simulink model "SimulinkFullblock"  (R2019b)
settings: Solver=VariableStepAuto  StartTime=0.0  StopTime=10  RelTol=1e-3
(part 2 of 5)

== matlab function SimulinkFullblock/Forward Acceleration  ==
  data: q input; pdd output; qd input; qdd input
function pdd    = fcn(q,qd,qdd)
q1= q(1);
q2= q(2);
q3= q(3);
q4= q(4);
q5= q(5);
q6= q(6);
q1d=qd(1);
q2d=qd(2);
q3d=qd(3);
q4d=qd(4);
q5d=qd(5);
q6d=qd(6);
q1dd= qdd(1);
q2dd= qdd(2);
q3dd= qdd(3);
q4dd= qdd(4);
q5dd= qdd(5);
q6dd= qdd(6);
L1=10;
L2=10;
L3=10;
L4=10;

Jdev= [ conj(L4)*(sin(0.0175*conj(q5) + 1.5708)*(0.0175*conj(q1d)*sin(0.0175*conj(q1) - 1.5708)*sin(0.0175*conj(q4) + 1.5708) - 0.0175*cos(0.0175*conj(q1) - 1.5708)*cos(0.0175*conj(q4) + 1.5708)*conj(q4d) - 0.0175*cos(0.0175*conj(q1) - 1.5708)*cos(0.0175*conj(q2) - 1.5708)*cos(0.0175*conj(q4) + 1.5708)*conj(q1d) + 0.0175*cos(0.0175*conj(q4) + 1.5708)*conj(q2d)*sin(0.0175*conj(q1) - 1.5708)*sin(0.0175*conj(q2) - 1.5708) + 0.0175*cos(0.0175*conj(q2) - 1.5708)*conj(q4d)*sin(0.0175*conj(q1) - 1.5708)*sin(0.0175*conj(q4) + 1.5708)) - 0.0175*cos(0.0175*conj(q5) + 1.5708)*conj(q5d)*(cos(0.0175*conj(q1) - 1.5708)*sin(0.0175*conj(q4) + 1.5708) + cos(0.0175*conj(q2) - 1.5708)*cos(0.0175*conj(q4) + 1.5708)*sin(0.0175*conj(q1) - 1.5708)) + 0.0175*cos(0.0175*conj(q1) - 1.5708)*cos(0.0175*conj(q5) + 1.5708)*conj(q1d)*sin(0.0175*conj(q2) - 1.5708) + 0.0175*cos(0.0175*conj(q2) - 1.5708)*cos(0.0175*conj(q5) + 1.5708)*conj(q2d)*sin(0.0175*conj(q1) - 1.5708) - 0.0175*conj(q5d)*sin(0.0175*conj(q1) - 1.5708)*sin(0.0175*conj(q2) - 1.5708)*sin(0.0175*conj(q5) + 1.5708)) - conj(q3d)*sin(0.0175*conj(q1) - 1.5708)*sin(0.0175*conj(q2) - 1.5708) - 0.0175*cos(0.0175*conj(q1) - 1.5708)*conj(q1d)*sin(0.0175*conj(q2) - 1.5708)*(conj(q3) + conj(L2)) - 0.0175*cos(0.0175*conj(q2) - 1.5708)*conj(q2d)*sin(0.0175*conj(q1) - 1.5708)*(conj(q3) + conj(L2)) - 0.0175*cos(0.0175*conj(q1) - 1.5708)*conj(q1d)*sin(0.0175*conj(q2) - 1.5708)*conj(L3) - 0.0175*cos(0.0175*conj(q2) - 1.5708)*conj(q2d)*sin(0.0175*conj(q1) - 1.5708)*conj(L3),                                                                                                                                                                                                                                                                                                                                                                                                                                                                                                                                                                                                                                                                                                                                                                                                                                                                                                                                                                                                                                                                                                                                                                                                                                                                                                                                                                                                                                                                                                                                                                                                                                                                                                                                                                                                                                                                                                                                                                                                                                                                                                                                                                                                                                                                                                                                                                                                                                                                                                                                                                                                                                                                                                                                                                                                                                                                                                                                                                                                                                                                                                                                                                                                                                                                                                                                                                                                                                                                                                                                                                                                                                                                                               cos(0.0175*conj(q1) - 1.5708)*(cos(0.0175*conj(q2) - 1.5708)*conj(q3d) + conj(L4)*(0.0175*cos(0.0175*conj(q5) + 1.5708)*conj(q2d)*sin(0.0175*conj(q2) - 1.5708) + 0.0175*cos(0.0175*conj(q2) - 1.5708)*conj(q5d)*sin(0.0175*conj(q5) + 1.5708) - 0.0175*cos(0.0175*conj(q2) - 1.5708)*cos(0.0175*conj(q4) + 1.5708)*conj(q2d)*sin(0.0175*conj(q5) + 1.5708) - 0.0175*cos(0.0175*conj(q4) + 1.5708)*cos(0.0175*conj(q5) + 1.5708)*conj(q5d)*sin(0.0175*conj(q2) - 1.5708) + 0.0175*conj(q4d)*sin(0.0175*conj(q2) - 1.5708)*sin(0.0175*conj(q4) + 1.5708)*sin(0.0175*conj(q5) + 1.5708)) - 0.0175*conj(q2d)*sin(0.0175*conj(q2) - 1.5708)*conj(L3) - 0.0175*conj(q2d)*sin(0.0175*conj(q2) - 1.5708)*(conj(q3) + conj(L2))) - 0.0175*conj(q1d)*sin(0.0175*conj(q1) - 1.5708)*(cos(0.0175*conj(q2) - 1.5708)*conj(L3) - conj(L4)*(cos(0.0175*conj(q2) - 1.5708)*cos(0.0175*conj(q5) + 1.5708) + cos(0.0175*conj(q4) + 1.5708)*sin(0.0175*conj(q2) - 1.5708)*sin(0.0175*conj(q5) + 1.5708)) + cos(0.0175*conj(q2) - 1.5708)*(conj(q3) + conj(L2))), 0.0175*cos(0.0175*q1 - 1.5708)*cos(0.0175*q2 - 1.5708)*q2d - 0.0175*sin(0.0175*q1 - 1.5708)*sin(0.0175*q2 - 1.5708)*q1d,                                                                                                                                                                                                                                                                                                                                                                                                                                                                                                                                                                                                                                                                                                                                                                                                                                                                                                                                                                                                                                                                                                                                                                                                                                                                                                                                                                                                                                                                                                                                                                                                                                                                                                                                                                                                                                                                                                                                                                                                                                                                                                                                                                                                                                                                                                                                                                                                                                                                          sin(0.0175*conj(q1) - 1.5708)*sin(0.0175*conj(q2) - 1.5708)*(cos(0.0175*conj(q2) - 1.5708)*conj(q3d) - cos(0.0175*conj(q2) - 1.5708)*conj(q3d) + conj(L4)*(0.0175*cos(0.0175*conj(q5) + 1.5708)*conj(q2d)*sin(0.0175*conj(q2) - 1.5708) + 0.0175*cos(0.0175*conj(q2) - 1.5708)*conj(q5d)*sin(0.0175*conj(q5) + 1.5708) - 0.0175*cos(0.0175*conj(q2) - 1.5708)*cos(0.0175*conj(q4) + 1.5708)*conj(q2d)*sin(0.0175*conj(q5) + 1.5708) - 0.0175*cos(0.0175*conj(q4) + 1.5708)*cos(0.0175*conj(q5) + 1.5708)*conj(q5d)*sin(0.0175*conj(q2) - 1.5708) + 0.0175*conj(q4d)*sin(0.0175*conj(q2) - 1.5708)*sin(0.0175*conj(q4) + 1.5708)*sin(0.0175*conj(q5) + 1.5708)) - 0.0175*conj(q2d)*sin(0.0175*conj(q2) - 1.5708)*conj(L3) - 0.0175*conj(q2d)*sin(0.0175*conj(q2) - 1.5708)*(conj(q3) + conj(L2)) + 0.0175*conj(q2d)*sin(0.0175*conj(q2) - 1.5708)*(conj(q3) + conj(L2))) - cos(0.0175*conj(q2) - 1.5708)*(conj(q3d)*sin(0.0175*conj(q1) - 1.5708)*sin(0.0175*conj(q2) - 1.5708) - conj(L4)*(sin(0.0175*conj(q5) + 1.5708)*(0.0175*conj(q1d)*sin(0.0175*conj(q1) - 1.5708)*sin(0.0175*conj(q4) + 1.5708) - 0.0175*cos(0.0175*conj(q1) - 1.5708)*cos(0.0175*conj(q4) + 1.5708)*conj(q4d) - 0.0175*cos(0.0175*conj(q1) - 1.5708)*cos(0.0175*conj(q2) - 1.5708)*cos(0.0175*conj(q4) + 1.5708)*conj(q1d) + 0.0175*cos(0.0175*conj(q4) + 1.5708)*conj(q2d)*sin(0.0175*conj(q1) - 1.5708)*sin(0.0175*conj(q2) - 1.5708) + 0.0175*cos(0.0175*conj(q2) - 1.5708)*conj(q4d)*sin(0.0175*conj(q1) - 1.5708)*sin(0.0175*conj(q4) + 1.5708)) - 0.0175*cos(0.0175*conj(q5) + 1.5708)*conj(q5d)*(cos(0.0175*conj(q1) - 1.5708)*sin(0.0175*conj(q4) + 1.5708) + cos(0.0175*conj(q2) - 1.5708)*cos(0.0175*conj(q4) + 1.5708)*sin(0.0175*conj(q1) - 1.5708)) + 0.0175*cos(0.0175*conj(q1) - 1.5708)*cos(0.0175*conj(q5) + 1.5708)*conj(q1d)*sin(0.0175*conj(q2) - 1.5708) + 0.0175*cos(0.0175*conj(q2) - 1.5708)*cos(0.0175*conj(q5) + 1.5708)*conj(q2d)*sin(0.0175*conj(q1) - 1.5708) - 0.0175*conj(q5d)*sin(0.0175*conj(q1) - 1.5708)*sin(0.0175*conj(q2) - 1.5708)*sin(0.0175*conj(q5) + 1.5708)) - conj(q3d)*sin(0.0175*conj(q1) - 1.5708)*sin(0.0175*conj(q2) - 1.5708) + 0.0175*cos(0.0175*conj(q1) - 1.5708)*conj(q1d)*sin(0.0175*conj(q2) - 1.5708)*(conj(q3) + conj(L2)) + 0.0175*cos(0.0175*conj(q2) - 1.5708)*conj(q2d)*sin(0.0175*conj(q1) - 1.5708)*(conj(q3) + conj(L2)) - 0.0175*cos(0.0175*conj(q1) - 1.5708)*conj(q1d)*sin(0.0175*conj(q2) - 1.5708)*(conj(q3) + conj(L2)) - 0.0175*cos(0.0175*conj(q2) - 1.5708)*conj(q2d)*sin(0.0175*conj(q1) - 1.5708)*(conj(q3) + conj(L2)) + 0.0175*cos(0.0175*conj(q1) - 1.5708)*conj(q1d)*sin(0.0175*conj(q2) - 1.5708)*conj(L3) + 0.0175*cos(0.0175*conj(q2) - 1.5708)*conj(q2d)*sin(0.0175*conj(q1) - 1.5708)*conj(L3)) + 0.0175*conj(q2d)*sin(0.0175*conj(q2) - 1.5708)*(conj(L4)*(sin(0.0175*conj(q5) + 1.5708)*(cos(0.0175*conj(q1) - 1.5708)*sin(0.0175*conj(q4) + 1.5708) + cos(0.0175*conj(q2) - 1.5708)*cos(0.0175*conj(q4) + 1.5708)*sin(0.0175*conj(q1) - 1.5708)) - cos(0.0175*conj(q5) + 1.5708)*sin(0.0175*conj(q1) - 1.5708)*sin(0.0175*conj(q2) - 1.5708)) + sin(0.0175*conj(q1) - 1.5708)*sin(0.0175*conj(q2) - 1.5708)*(conj(q3) + conj(L2)) - sin(0.0175*conj(q1) - 1.5708)*sin(0.0175*conj(q2) - 1.5708)*(conj(q3) + conj(L2)) + sin(0.0175*conj(q1) - 1.5708)*sin(0.0175*conj(q2) - 1.5708)*conj(L3)) + 0.0175*cos(0.0175*conj(q1) - 1.5708)*conj(q1d)*sin(0.0175*conj(q2) - 1.5708)*(cos(0.0175*conj(q2) - 1.5708)*conj(L3) - conj(L4)*(cos(0.0175*conj(q2) - 1.5708)*cos(0.0175*conj(q5) + 1.5708) + cos(0.0175*conj(q4) + 1.5708)*sin(0.0175*conj(q2) - 1.5708)*sin(0.0175*conj(q5) + 1.5708)) + cos(0.0175*conj(q2) - 1.5708)*(conj(q3) + conj(L2)) - cos(0.0175*conj(q2) - 1.5708)*(conj(q3) + conj(L2))) + 0.0175*cos(0.0175*conj(q2) - 1.5708)*conj(q2d)*sin(0.0175*conj(q1) - 1.5708)*(cos(0.0175*conj(q2) - 1.5708)*conj(L3) - conj(L4)*(cos(0.0175*conj(q2) - 1.5708)*cos(0.0175*conj(q5) + 1.5708) + cos(0.0175*conj(q4) + 1.5708)*sin(0.0175*conj(q2) - 1.5708)*sin(0.0175*conj(q5) + 1.5708)) + cos(0.0175*conj(q2) - 1.5708)*(conj(q3) + conj(L2)) - cos(0.0175*conj(q2) - 1.5708)*(conj(q3) + conj(L2))),                                                                                                                                                                                                                                                                                                                                                                                                                                                                                                                                                                                                                                                                                                                                                                                                                                                                                                                                                                                                                                                                                                                                                                                                                                                                                                                                                                                                                                                                 0.0175*cos(0.0175*conj(q2) - 1.5708)*conj(q2d)*sin(0.0175*conj(q4) + 1.5708)*(conj(L4)*(sin(0.0175*conj(q5) + 1.5708)*(cos(0.0175*conj(q1) - 1.5708)*sin(0.0175*conj(q4) + 1.5708) + cos(0.0175*conj(q2) - 1.5708)*cos(0.0175*conj(q4) + 1.5708)*sin(0.0175*conj(q1) - 1.5708)) - cos(0.0175*conj(q5) + 1.5708)*sin(0.0175*conj(q1) - 1.5708)*sin(0.0175*conj(q2) - 1.5708)) + sin(0.0175*conj(q1) - 1.5708)*sin(0.0175*conj(q2) - 1.5708)*(conj(q3) + conj(L2)) - sin(0.0175*conj(q1) - 1.5708)*sin(0.0175*conj(q2) - 1.5708)*(conj(q3) + conj(L2)) + sin(0.0175*conj(q1) - 1.5708)*sin(0.0175*conj(q2) - 1.5708)*conj(L3) - sin(0.0175*conj(q1) - 1.5708)*sin(0.0175*conj(q2) - 1.5708)*conj(L3)) - (cos(0.0175*conj(q1) - 1.5708)*cos(0.0175*conj(q4) + 1.5708) - cos(0.0175*conj(q2) - 1.5708)*sin(0.0175*conj(q1) - 1.5708)*sin(0.0175*conj(q4) + 1.5708))*(cos(0.0175*conj(q2) - 1.5708)*conj(q3d) - cos(0.0175*conj(q2) - 1.5708)*conj(q3d) + conj(L4)*(0.0175*cos(0.0175*conj(q5) + 1.5708)*conj(q2d)*sin(0.0175*conj(q2) - 1.5708) + 0.0175*cos(0.0175*conj(q2) - 1.5708)*conj(q5d)*sin(0.0175*conj(q5) + 1.5708) - 0.0175*cos(0.0175*conj(q2) - 1.5708)*cos(0.0175*conj(q4) + 1.5708)*conj(q2d)*sin(0.0175*conj(q5) + 1.5708) - 0.0175*cos(0.0175*conj(q4) + 1.5708)*cos(0.0175*conj(q5) + 1.5708)*conj(q5d)*sin(0.0175*conj(q2) - 1.5708) + 0.0175*conj(q4d)*sin(0.0175*conj(q2) - 1.5708)*sin(0.0175*conj(q4) + 1.5708)*sin(0.0175*conj(q5) + 1.5708)) - 0.0175*conj(q2d)*sin(0.0175*conj(q2) - 1.5708)*conj(L3) + 0.0175*conj(q2d)*sin(0.0175*conj(q2) - 1.5708)*conj(L3) - 0.0175*conj(q2d)*sin(0.0175*conj(q2) - 1.5708)*(conj(q3) + conj(L2)) + 0.0175*conj(q2d)*sin(0.0175*conj(q2) - 1.5708)*(conj(q3) + conj(L2))) - sin(0.0175*conj(q2) - 1.5708)*sin(0.0175*conj(q4) + 1.5708)*(conj(L4)*(sin(0.0175*conj(q5) + 1.5708)*(0.0175*conj(q1d)*sin(0.0175*conj(q1) - 1.5708)*sin(0.0175*conj(q4) + 1.5708) - 0.0175*cos(0.0175*conj(q1) - 1.5708)*cos(0.0175*conj(q4) + 1.5708)*conj(q4d) - 0.0175*cos(0.0175*conj(q1) - 1.5708)*cos(0.0175*conj(q2) - 1.5708)*cos(0.0175*conj(q4) + 1.5708)*conj(q1d) + 0.0175*cos(0.0175*conj(q4) + 1.5708)*conj(q2d)*sin(0.0175*conj(q1) - 1.5708)*sin(0.0175*conj(q2) - 1.5708) + 0.0175*cos(0.0175*conj(q2) - 1.5708)*conj(q4d)*sin(0.0175*conj(q1) - 1.5708)*sin(0.0175*conj(q4) + 1.5708)) - 0.0175*cos(0.0175*conj(q5) + 1.5708)*conj(q5d)*(cos(0.0175*conj(q1) - 1.5708)*sin(0.0175*conj(q4) + 1.5708) + cos(0.0175*conj(q2) - 1.5708)*cos(0.0175*conj(q4) + 1.5708)*sin(0.0175*conj(q1) - 1.5708)) + 0.0175*cos(0.0175*conj(q1) - 1.5708)*cos(0.0175*conj(q5) + 1.5708)*conj(q1d)*sin(0.0175*conj(q2) - 1.5708) + 0.0175*cos(0.0175*conj(q2) - 1.5708)*cos(0.0175*conj(q5) + 1.5708)*conj(q2d)*sin(0.0175*conj(q1) - 1.5708) - 0.0175*conj(q5d)*sin(0.0175*conj(q1) - 1.5708)*sin(0.0175*conj(q2) - 1.5708)*sin(0.0175*conj(q5) + 1.5708)) - conj(q3d)*sin(0.0175*conj(q1) - 1.5708)*sin(0.0175*conj(q2) - 1.5708) + conj(q3d)*sin(0.0175*conj(q1) - 1.5708)*sin(0.0175*conj(q2) - 1.5708) - 0.0175*cos(0.0175*conj(q1) - 1.5708)*conj(q1d)*sin(0.0175*conj(q2) - 1.5708)*(conj(q3) + conj(L2)) - 0.0175*cos(0.0175*conj(q2) - 1.5708)*conj(q2d)*sin(0.0175*conj(q1) - 1.5708)*(conj(q3) + conj(L2)) + 0.0175*cos(0.0175*conj(q1) - 1.5708)*conj(q1d)*sin(0.0175*conj(q2) - 1.5708)*(conj(q3) + conj(L2)) + 0.0175*cos(0.0175*conj(q2) - 1.5708)*conj(q2d)*sin(0.0175*conj(q1) - 1.5708)*(conj(q3) + conj(L2)) - 0.0175*cos(0.0175*conj(q1) - 1.5708)*conj(q1d)*sin(0.0175*conj(q2) - 1.5708)*conj(L3) - 0.0175*cos(0.0175*conj(q2) - 1.5708)*conj(q2d)*sin(0.0175*conj(q1) - 1.5708)*conj(L3) + 0.0175*cos(0.0175*conj(q1) - 1.5708)*conj(q1d)*sin(0.0175*conj(q2) - 1.5708)*conj(L3) + 0.0175*cos(0.0175*conj(q2) - 1.5708)*conj(q2d)*sin(0.0175*conj(q1) - 1.5708)*conj(L3)) - (cos(0.0175*conj(q2) - 1.5708)*conj(L3) - cos(0.0175*conj(q2) - 1.5708)*conj(L3) + conj(L4)*(cos(0.0175*conj(q2) - 1.5708)*cos(0.0175*conj(q5) + 1.5708) + cos(0.0175*conj(q4) + 1.5708)*sin(0.0175*conj(q2) - 1.5708)*sin(0.0175*conj(q5) + 1.5708)) - cos(0.0175*conj(q2) - 1.5708)*(conj(q3) + conj(L2)) + cos(0.0175*conj(q2) - 1.5708)*(conj(q3) + conj(L2)))*(0.0175*cos(0.0175*conj(q4) + 1.5708)*conj(q1d)*sin(0.0175*conj(q1) - 1.5708) + 0.0175*cos(0.0175*conj(q1) - 1.5708)*conj(q4d)*sin(0.0175*conj(q4) + 1.5708) + 0.0175*cos(0.0175*conj(q1) - 1.5708)*cos(0.0175*conj(q2) - 1.5708)*conj(q1d)*sin(0.0175*conj(q4) + 1.5708) + 0.0175*cos(0.0175*conj(q2) - 1.5708)*cos(0.0175*conj(q4) + 1.5708)*conj(q4d)*sin(0.0175*conj(q1) - 1.5708) - 0.0175*conj(q2d)*sin(0.0175*conj(q1) - 1.5708)*sin(0.0175*conj(q2) - 1.5708)*sin(0.0175*conj(q4) + 1.5708)) + 0.0175*cos(0.0175*conj(q4) + 1.5708)*conj(q4d)*sin(0.0175*conj(q2) - 1.5708)*(conj(L4)*(sin(0.0175*conj(q5) + 1.5708)*(cos(0.0175*conj(q1) - 1.5708)*sin(0.0175*conj(q4) + 1.5708) + cos(0.0175*conj(q2) - 1.5708)*cos(0.0175*conj(q4) + 1.5708)*sin(0.0175*conj(q1) - 1.5708)) - cos(0.0175*conj(q5) + 1.5708)*sin(0.0175*conj(q1) - 1.5708)*sin(0.0175*conj(q2) - 1.5708)) + sin(0.0175*conj(q1) - 1.5708)*sin(0.0175*conj(q2) - 1.5708)*(conj(q3) + conj(L2)) - sin(0.0175*conj(q1) - 1.5708)*sin(0.0175*conj(q2) - 1.5708)*(conj(q3) + conj(L2)) + sin(0.0175*conj(q1) - 1.5708)*sin(0.0175*conj(q2) - 1.5708)*conj(L3) - sin(0.0175*conj(q1) - 1.5708)*sin(0.0175*conj(q2) - 1.5708)*conj(L3)),                                                                                                                                                                                                                                                                                                                                                                                                                                                                                                                                                                                                                                                                                                                                                                                                                                                                                                                                                                                                                                                                                                                                                                                                                                                                                                                                                                                                                                                                                                                                                                                                                                                                                                                                                                                                                                                                                                                                                                                                                                                                                                                                                                                                                                                                                                                                                                                                                                                           (cos(0.0175*conj(q2) - 1.5708)*conj(L3) - cos(0.0175*conj(q2) - 1.5708)*conj(L3) + conj(L4)*(cos(0.0175*conj(q2) - 1.5708)*cos(0.0175*conj(q5) + 1.5708) + cos(0.0175*conj(q4) + 1.5708)*sin(0.0175*conj(q2) - 1.5708)*sin(0.0175*conj(q5) + 1.5708)) - cos(0.0175*conj(q2) - 1.5708)*(conj(q3) + conj(L2)) + cos(0.0175*conj(q2) - 1.5708)*(conj(q3) + conj(L2)))*(sin(0.0175*conj(q5) + 1.5708)*(0.0175*conj(q1d)*sin(0.0175*conj(q1) - 1.5708)*sin(0.0175*conj(q4) + 1.5708) - 0.0175*cos(0.0175*conj(q1) - 1.5708)*cos(0.0175*conj(q4) + 1.5708)*conj(q4d) - 0.0175*cos(0.0175*conj(q1) - 1.5708)*cos(0.0175*conj(q2) - 1.5708)*cos(0.0175*conj(q4) + 1.5708)*conj(q1d) + 0.0175*cos(0.0175*conj(q4) + 1.5708)*conj(q2d)*sin(0.0175*conj(q1) - 1.5708)*sin(0.0175*conj(q2) - 1.5708) + 0.0175*cos(0.0175*conj(q2) - 1.5708)*conj(q4d)*sin(0.0175*conj(q1) - 1.5708)*sin(0.0175*conj(q4) + 1.5708)) - 0.0175*cos(0.0175*conj(q5) + 1.5708)*conj(q5d)*(cos(0.0175*conj(q1) - 1.5708)*sin(0.0175*conj(q4) + 1.5708) + cos(0.0175*conj(q2) - 1.5708)*cos(0.0175*conj(q4) + 1.5708)*sin(0.0175*conj(q1) - 1.5708)) + 0.0175*cos(0.0175*conj(q1) - 1.5708)*cos(0.0175*conj(q5) + 1.5708)*conj(q1d)*sin(0.0175*conj(q2) - 1.5708) + 0.0175*cos(0.0175*conj(q2) - 1.5708)*cos(0.0175*conj(q5) + 1.5708)*conj(q2d)*sin(0.0175*conj(q1) - 1.5708) - 0.0175*conj(q5d)*sin(0.0175*conj(q1) - 1.5708)*sin(0.0175*conj(q2) - 1.5708)*sin(0.0175*conj(q5) + 1.5708)) - (cos(0.0175*conj(q2) - 1.5708)*cos(0.0175*conj(q5) + 1.5708) + cos(0.0175*conj(q4) + 1.5708)*sin(0.0175*conj(q2) - 1.5708)*sin(0.0175*conj(q5) + 1.5708))*(conj(L4)*(sin(0.0175*conj(q5) + 1.5708)*(0.0175*conj(q1d)*sin(0.0175*conj(q1) - 1.5708)*sin(0.0175*conj(q4) + 1.5708) - 0.0175*cos(0.0175*conj(q1) - 1.5708)*cos(0.0175*conj(q4) + 1.5708)*conj(q4d) - 0.0175*cos(0.0175*conj(q1) - 1.5708)*cos(0.0175*conj(q2) - 1.5708)*cos(0.0175*conj(q4) + 1.5708)*conj(q1d) + 0.0175*cos(0.0175*conj(q4) + 1.5708)*conj(q2d)*sin(0.0175*conj(q1) - 1.5708)*sin(0.0175*conj(q2) - 1.5708) + 0.0175*cos(0.0175*conj(q2) - 1.5708)*conj(q4d)*sin(0.0175*conj(q1) - 1.5708)*sin(0.0175*conj(q4) + 1.5708)) - 0.0175*cos(0.0175*conj(q5) + 1.5708)*conj(q5d)*(cos(0.0175*conj(q1) - 1.5708)*sin(0.0175*conj(q4) + 1.5708) + cos(0.0175*conj(q2) - 1.5708)*cos(0.0175*conj(q4) + 1.5708)*sin(0.0175*conj(q1) - 1.5708)) + 0.0175*cos(0.0175*conj(q1) - 1.5708)*cos(0.0175*conj(q5) + 1.5708)*conj(q1d)*sin(0.0175*conj(q2) - 1.5708) + 0.0175*cos(0.0175*conj(q2) - 1.5708)*cos(0.0175*conj(q5) + 1.5708)*conj(q2d)*sin(0.0175*conj(q1) - 1.5708) - 0.0175*conj(q5d)*sin(0.0175*conj(q1) - 1.5708)*sin(0.0175*conj(q2) - 1.5708)*sin(0.0175*conj(q5) + 1.5708)) - conj(q3d)*sin(0.0175*conj(q1) - 1.5708)*sin(0.0175*conj(q2) - 1.5708) + conj(q3d)*sin(0.0175*conj(q1) - 1.5708)*sin(0.0175*conj(q2) - 1.5708) - 0.0175*cos(0.0175*conj(q1) - 1.5708)*conj(q1d)*sin(0.0175*conj(q2) - 1.5708)*(conj(q3) + conj(L2)) - 0.0175*cos(0.0175*conj(q2) - 1.5708)*conj(q2d)*sin(0.0175*conj(q1) - 1.5708)*(conj(q3) + conj(L2)) + 0.0175*cos(0.0175*conj(q1) - 1.5708)*conj(q1d)*sin(0.0175*conj(q2) - 1.5708)*(conj(q3) + conj(L2)) + 0.0175*cos(0.0175*conj(q2) - 1.5708)*conj(q2d)*sin(0.0175*conj(q1) - 1.5708)*(conj(q3) + conj(L2)) - 0.0175*cos(0.0175*conj(q1) - 1.5708)*conj(q1d)*sin(0.0175*conj(q2) - 1.5708)*conj(L3) - 0.0175*cos(0.0175*conj(q2) - 1.5708)*conj(q2d)*sin(0.0175*conj(q1) - 1.5708)*conj(L3) + 0.0175*cos(0.0175*conj(q1) - 1.5708)*conj(q1d)*sin(0.0175*conj(q2) - 1.5708)*conj(L3) + 0.0175*cos(0.0175*conj(q2) - 1.5708)*conj(q2d)*sin(0.0175*conj(q1) - 1.5708)*conj(L3)) - (conj(L4)*(sin(0.0175*conj(q5) + 1.5708)*(cos(0.0175*conj(q1) - 1.5708)*sin(0.0175*conj(q4) + 1.5708) + cos(0.0175*conj(q2) - 1.5708)*cos(0.0175*conj(q4) + 1.5708)*sin(0.0175*conj(q1) - 1.5708)) - cos(0.0175*conj(q5) + 1.5708)*sin(0.0175*conj(q1) - 1.5708)*sin(0.0175*conj(q2) - 1.5708)) + sin(0.0175*conj(q1) - 1.5708)*sin(0.0175*conj(q2) - 1.5708)*(conj(q3) + conj(L2)) - sin(0.0175*conj(q1) - 1.5708)*sin(0.0175*conj(q2) - 1.5708)*(conj(q3) + conj(L2)) + sin(0.0175*conj(q1) - 1.5708)*sin(0.0175*conj(q2) - 1.5708)*conj(L3) - sin(0.0175*conj(q1) - 1.5708)*sin(0.0175*conj(q2) - 1.5708)*conj(L3))*(0.0175*cos(0.0175*conj(q5) + 1.5708)*conj(q2d)*sin(0.0175*conj(q2) - 1.5708) + 0.0175*cos(0.0175*conj(q2) - 1.5708)*conj(q5d)*sin(0.0175*conj(q5) + 1.5708) - 0.0175*cos(0.0175*conj(q2) - 1.5708)*cos(0.0175*conj(q4) + 1.5708)*conj(q2d)*sin(0.0175*conj(q5) + 1.5708) - 0.0175*cos(0.0175*conj(q4) + 1.5708)*cos(0.0175*conj(q5) + 1.5708)*conj(q5d)*sin(0.0175*conj(q2) - 1.5708) + 0.0175*conj(q4d)*sin(0.0175*conj(q2) - 1.5708)*sin(0.0175*conj(q4) + 1.5708)*sin(0.0175*conj(q5) + 1.5708)) + (sin(0.0175*conj(q5) + 1.5708)*(cos(0.0175*conj(q1) - 1.5708)*sin(0.0175*conj(q4) + 1.5708) + cos(0.0175*conj(q2) - 1.5708)*cos(0.0175*conj(q4) + 1.5708)*sin(0.0175*conj(q1) - 1.5708)) - cos(0.0175*conj(q5) + 1.5708)*sin(0.0175*conj(q1) - 1.5708)*sin(0.0175*conj(q2) - 1.5708))*(cos(0.0175*conj(q2) - 1.5708)*conj(q3d) - cos(0.0175*conj(q2) - 1.5708)*conj(q3d) + conj(L4)*(0.0175*cos(0.0175*conj(q5) + 1.5708)*conj(q2d)*sin(0.0175*conj(q2) - 1.5708) + 0.0175*cos(0.0175*conj(q2) - 1.5708)*conj(q5d)*sin(0.0175*conj(q5) + 1.5708) - 0.0175*cos(0.0175*conj(q2) - 1.5708)*cos(0.0175*conj(q4) + 1.5708)*conj(q2d)*sin(0.0175*conj(q5) + 1.5708) - 0.0175*cos(0.0175*conj(q4) + 1.5708)*cos(0.0175*conj(q5) + 1.5708)*conj(q5d)*sin(0.0175*conj(q2) - 1.5708) + 0.0175*conj(q4d)*sin(0.0175*conj(q2) - 1.5708)*sin(0.0175*conj(q4) + 1.5708)*sin(0.0175*conj(q5) + 1.5708)) - 0.0175*conj(q2d)*sin(0.0175*conj(q2) - 1.5708)*conj(L3) + 0.0175*conj(q2d)*sin(0.0175*conj(q2) - 1.5708)*conj(L3) - 0.0175*conj(q2d)*sin(0.0175*conj(q2) - 1.5708)*(conj(q3) + conj(L2)) + 0.0175*conj(q2d)*sin(0.0175*conj(q2) - 1.5708)*(conj(q3) + conj(L2)));
 cos(0.0175*conj(q1) - 1.5708)*conj(q3d)*sin(0.0175*conj(q2) - 1.5708) - conj(L4)*(sin(0.0175*conj(q5) + 1.5708)*(0.0175*cos(0.0175*conj(q1) - 1.5708)*conj(q1d)*sin(0.0175*conj(q4) + 1.5708) + 0.0175*cos(0.0175*conj(q4) + 1.5708)*conj(q4d)*sin(0.0175*conj(q1) - 1.5708) + 0.0175*cos(0.0175*conj(q2) - 1.5708)*cos(0.0175*conj(q4) + 1.5708)*conj(q1d)*sin(0.0175*conj(q1) - 1.5708) + 0.0175*cos(0.0175*conj(q1) - 1.5708)*cos(0.0175*conj(q4) + 1.5708)*conj(q2d)*sin(0.0175*conj(q2) - 1.5708) + 0.0175*cos(0.0175*conj(q1) - 1.5708)*cos(0.0175*conj(q2) - 1.5708)*conj(q4d)*sin(0.0175*conj(q4) + 1.5708)) + 0.0175*cos(0.0175*conj(q5) + 1.5708)*conj(q5d)*(sin(0.0175*conj(q1) - 1.5708)*sin(0.0175*conj(q4) + 1.5708) - cos(0.0175*conj(q1) - 1.5708)*cos(0.0175*conj(q2) - 1.5708)*cos(0.0175*conj(q4) + 1.5708)) + 0.0175*cos(0.0175*conj(q1) - 1.5708)*cos(0.0175*conj(q2) - 1.5708)*cos(0.0175*conj(q5) + 1.5708)*conj(q2d) - 0.0175*cos(0.0175*conj(q5) + 1.5708)*conj(q1d)*sin(0.0175*conj(q1) - 1.5708)*sin(0.0175*conj(q2) - 1.5708) - 0.0175*cos(0.0175*conj(q1) - 1.5708)*conj(q5d)*sin(0.0175*conj(q2) - 1.5708)*sin(0.0175*conj(q5) + 1.5708)) + 0.0175*cos(0.0175*conj(q1) - 1.5708)*cos(0.0175*conj(q2) - 1.5708)*conj(q2d)*(conj(q3) + conj(L2)) - 0.0175*conj(q1d)*sin(0.0175*conj(q1) - 1.5708)*sin(0.0175*conj(q2) - 1.5708)*(conj(q3) + conj(L2)) + 0.0175*cos(0.0175*conj(q1) - 1.5708)*cos(0.0175*conj(q2) - 1.5708)*conj(q2d)*conj(L3) - 0.0175*conj(q1d)*sin(0.0175*conj(q1) - 1.5708)*sin(0.0175*conj(q2) - 1.5708)*conj(L3),                                                                                                                                                                                                                                                                                                                                                                                                                                                                                                                                                                                                                                                                                                                                                                                                                                                                                                                                                                                                                                                                                                                                                                                                                                                                                                                                                                                                                                                                                                                                                                                                                                                                                                                                                                                                                                                                                                                                                                                                                                                                                                                                                                                                                                                                                                                                                                                                                                                                                                                                                                                                                                                                                                                                                                                                                                                                                                                                                                                                                                                                                                                                                                                                                                                                                                                                                                                                                                                                                                                                                                                                                                                                                               sin(0.0175*conj(q1) - 1.5708)*(cos(0.0175*conj(q2) - 1.5708)*conj(q3d) + conj(L4)*(0.0175*cos(0.0175*conj(q5) + 1.5708)*conj(q2d)*sin(0.0175*conj(q2) - 1.5708) + 0.0175*cos(0.0175*conj(q2) - 1.5708)*conj(q5d)*sin(0.0175*conj(q5) + 1.5708) - 0.0175*cos(0.0175*conj(q2) - 1.5708)*cos(0.0175*conj(q4) + 1.5708)*conj(q2d)*sin(0.0175*conj(q5) + 1.5708) - 0.0175*cos(0.0175*conj(q4) + 1.5708)*cos(0.0175*conj(q5) + 1.5708)*conj(q5d)*sin(0.0175*conj(q2) - 1.5708) + 0.0175*conj(q4d)*sin(0.0175*conj(q2) - 1.5708)*sin(0.0175*conj(q4) + 1.5708)*sin(0.0175*conj(q5) + 1.5708)) - 0.0175*conj(q2d)*sin(0.0175*conj(q2) - 1.5708)*conj(L3) - 0.0175*conj(q2d)*sin(0.0175*conj(q2) - 1.5708)*(conj(q3) + conj(L2))) + 0.0175*cos(0.0175*conj(q1) - 1.5708)*conj(q1d)*(cos(0.0175*conj(q2) - 1.5708)*conj(L3) - conj(L4)*(cos(0.0175*conj(q2) - 1.5708)*cos(0.0175*conj(q5) + 1.5708) + cos(0.0175*conj(q4) + 1.5708)*sin(0.0175*conj(q2) - 1.5708)*sin(0.0175*conj(q5) + 1.5708)) + cos(0.0175*conj(q2) - 1.5708)*(conj(q3) + conj(L2))), 0.0175*cos(0.0175*q1 - 1.5708)*sin(0.0175*q2 - 1.5708)*q1d + 0.0175*cos(0.0175*q2 - 1.5708)*sin(0.0175*q1 - 1.5708)*q2d,                                                                                                                                                                                                                                                                                                                                                                                                                                                                                                                                                                                                                                                                                                                                                                                                                                                                                                                                                                                                                                                                                                                                                                                                                                                                                                                                                                                                                                                                                                                                                                                                                                                                                                                                                                                                                                                                                                                                                                                                                                                                                                                                                                                                                                                                                                                                                                                                                                                                          0.0175*conj(q2d)*sin(0.0175*conj(q2) - 1.5708)*(conj(L4)*(sin(0.0175*conj(q5) + 1.5708)*(sin(0.0175*conj(q1) - 1.5708)*sin(0.0175*conj(q4) + 1.5708) - cos(0.0175*conj(q1) - 1.5708)*cos(0.0175*conj(q2) - 1.5708)*cos(0.0175*conj(q4) + 1.5708)) + cos(0.0175*conj(q1) - 1.5708)*cos(0.0175*conj(q5) + 1.5708)*sin(0.0175*conj(q2) - 1.5708)) - cos(0.0175*conj(q1) - 1.5708)*sin(0.0175*conj(q2) - 1.5708)*conj(L3) - cos(0.0175*conj(q1) - 1.5708)*sin(0.0175*conj(q2) - 1.5708)*(conj(q3) + conj(L2)) + cos(0.0175*conj(q1) - 1.5708)*sin(0.0175*conj(q2) - 1.5708)*(conj(q3) + conj(L2))) - cos(0.0175*conj(q1) - 1.5708)*sin(0.0175*conj(q2) - 1.5708)*(cos(0.0175*conj(q2) - 1.5708)*conj(q3d) - cos(0.0175*conj(q2) - 1.5708)*conj(q3d) + conj(L4)*(0.0175*cos(0.0175*conj(q5) + 1.5708)*conj(q2d)*sin(0.0175*conj(q2) - 1.5708) + 0.0175*cos(0.0175*conj(q2) - 1.5708)*conj(q5d)*sin(0.0175*conj(q5) + 1.5708) - 0.0175*cos(0.0175*conj(q2) - 1.5708)*cos(0.0175*conj(q4) + 1.5708)*conj(q2d)*sin(0.0175*conj(q5) + 1.5708) - 0.0175*cos(0.0175*conj(q4) + 1.5708)*cos(0.0175*conj(q5) + 1.5708)*conj(q5d)*sin(0.0175*conj(q2) - 1.5708) + 0.0175*conj(q4d)*sin(0.0175*conj(q2) - 1.5708)*sin(0.0175*conj(q4) + 1.5708)*sin(0.0175*conj(q5) + 1.5708)) - 0.0175*conj(q2d)*sin(0.0175*conj(q2) - 1.5708)*conj(L3) - 0.0175*conj(q2d)*sin(0.0175*conj(q2) - 1.5708)*(conj(q3) + conj(L2)) + 0.0175*conj(q2d)*sin(0.0175*conj(q2) - 1.5708)*(conj(q3) + conj(L2))) - cos(0.0175*conj(q2) - 1.5708)*(conj(L4)*(sin(0.0175*conj(q5) + 1.5708)*(0.0175*cos(0.0175*conj(q1) - 1.5708)*conj(q1d)*sin(0.0175*conj(q4) + 1.5708) + 0.0175*cos(0.0175*conj(q4) + 1.5708)*conj(q4d)*sin(0.0175*conj(q1) - 1.5708) + 0.0175*cos(0.0175*conj(q2) - 1.5708)*cos(0.0175*conj(q4) + 1.5708)*conj(q1d)*sin(0.0175*conj(q1) - 1.5708) + 0.0175*cos(0.0175*conj(q1) - 1.5708)*cos(0.0175*conj(q4) + 1.5708)*conj(q2d)*sin(0.0175*conj(q2) - 1.5708) + 0.0175*cos(0.0175*conj(q1) - 1.5708)*cos(0.0175*conj(q2) - 1.5708)*conj(q4d)*sin(0.0175*conj(q4) + 1.5708)) + 0.0175*cos(0.0175*conj(q5) + 1.5708)*conj(q5d)*(sin(0.0175*conj(q1) - 1.5708)*sin(0.0175*conj(q4) + 1.5708) - cos(0.0175*conj(q1) - 1.5708)*cos(0.0175*conj(q2) - 1.5708)*cos(0.0175*conj(q4) + 1.5708)) + 0.0175*cos(0.0175*conj(q1) - 1.5708)*cos(0.0175*conj(q2) - 1.5708)*cos(0.0175*conj(q5) + 1.5708)*conj(q2d) - 0.0175*cos(0.0175*conj(q5) + 1.5708)*conj(q1d)*sin(0.0175*conj(q1) - 1.5708)*sin(0.0175*conj(q2) - 1.5708) - 0.0175*cos(0.0175*conj(q1) - 1.5708)*conj(q5d)*sin(0.0175*conj(q2) - 1.5708)*sin(0.0175*conj(q5) + 1.5708)) - cos(0.0175*conj(q1) - 1.5708)*conj(q3d)*sin(0.0175*conj(q2) - 1.5708) + cos(0.0175*conj(q1) - 1.5708)*conj(q3d)*sin(0.0175*conj(q2) - 1.5708) - 0.0175*cos(0.0175*conj(q1) - 1.5708)*cos(0.0175*conj(q2) - 1.5708)*conj(q2d)*(conj(q3) + conj(L2)) + 0.0175*cos(0.0175*conj(q1) - 1.5708)*cos(0.0175*conj(q2) - 1.5708)*conj(q2d)*(conj(q3) + conj(L2)) + 0.0175*conj(q1d)*sin(0.0175*conj(q1) - 1.5708)*sin(0.0175*conj(q2) - 1.5708)*(conj(q3) + conj(L2)) - 0.0175*conj(q1d)*sin(0.0175*conj(q1) - 1.5708)*sin(0.0175*conj(q2) - 1.5708)*(conj(q3) + conj(L2)) - 0.0175*cos(0.0175*conj(q1) - 1.5708)*cos(0.0175*conj(q2) - 1.5708)*conj(q2d)*conj(L3) + 0.0175*conj(q1d)*sin(0.0175*conj(q1) - 1.5708)*sin(0.0175*conj(q2) - 1.5708)*conj(L3)) - 0.0175*cos(0.0175*conj(q1) - 1.5708)*cos(0.0175*conj(q2) - 1.5708)*conj(q2d)*(cos(0.0175*conj(q2) - 1.5708)*conj(L3) - conj(L4)*(cos(0.0175*conj(q2) - 1.5708)*cos(0.0175*conj(q5) + 1.5708) + cos(0.0175*conj(q4) + 1.5708)*sin(0.0175*conj(q2) - 1.5708)*sin(0.0175*conj(q5) + 1.5708)) + cos(0.0175*conj(q2) - 1.5708)*(conj(q3) + conj(L2)) - cos(0.0175*conj(q2) - 1.5708)*(conj(q3) + conj(L2))) + 0.0175*conj(q1d)*sin(0.0175*conj(q1) - 1.5708)*sin(0.0175*conj(q2) - 1.5708)*(cos(0.0175*conj(q2) - 1.5708)*conj(L3) - conj(L4)*(cos(0.0175*conj(q2) - 1.5708)*cos(0.0175*conj(q5) + 1.5708) + cos(0.0175*conj(q4) + 1.5708)*sin(0.0175*conj(q2) - 1.5708)*sin(0.0175*conj(q5) + 1.5708)) + cos(0.0175*conj(q2) - 1.5708)*(conj(q3) + conj(L2)) - cos(0.0175*conj(q2) - 1.5708)*(conj(q3) + conj(L2))),                                                                                                                                                                                                                                                                                                                                                                                                                                                                                                                                                                                                                                                                                                                                                                                                                                                                                                                                                                                                                                                                                                                                                                                                                                                                                                                                                                                                                                                                 sin(0.0175*conj(q2) - 1.5708)*sin(0.0175*conj(q4) + 1.5708)*(conj(L4)*(sin(0.0175*conj(q5) + 1.5708)*(0.0175*cos(0.0175*conj(q1) - 1.5708)*conj(q1d)*sin(0.0175*conj(q4) + 1.5708) + 0.0175*cos(0.0175*conj(q4) + 1.5708)*conj(q4d)*sin(0.0175*conj(q1) - 1.5708) + 0.0175*cos(0.0175*conj(q2) - 1.5708)*cos(0.0175*conj(q4) + 1.5708)*conj(q1d)*sin(0.0175*conj(q1) - 1.5708) + 0.0175*cos(0.0175*conj(q1) - 1.5708)*cos(0.0175*conj(q4) + 1.5708)*conj(q2d)*sin(0.0175*conj(q2) - 1.5708) + 0.0175*cos(0.0175*conj(q1) - 1.5708)*cos(0.0175*conj(q2) - 1.5708)*conj(q4d)*sin(0.0175*conj(q4) + 1.5708)) + 0.0175*cos(0.0175*conj(q5) + 1.5708)*conj(q5d)*(sin(0.0175*conj(q1) - 1.5708)*sin(0.0175*conj(q4) + 1.5708) - cos(0.0175*conj(q1) - 1.5708)*cos(0.0175*conj(q2) - 1.5708)*cos(0.0175*conj(q4) + 1.5708)) + 0.0175*cos(0.0175*conj(q1) - 1.5708)*cos(0.0175*conj(q2) - 1.5708)*cos(0.0175*conj(q5) + 1.5708)*conj(q2d) - 0.0175*cos(0.0175*conj(q5) + 1.5708)*conj(q1d)*sin(0.0175*conj(q1) - 1.5708)*sin(0.0175*conj(q2) - 1.5708) - 0.0175*cos(0.0175*conj(q1) - 1.5708)*conj(q5d)*sin(0.0175*conj(q2) - 1.5708)*sin(0.0175*conj(q5) + 1.5708)) - cos(0.0175*conj(q1) - 1.5708)*conj(q3d)*sin(0.0175*conj(q2) - 1.5708) + cos(0.0175*conj(q1) - 1.5708)*conj(q3d)*sin(0.0175*conj(q2) - 1.5708) - 0.0175*cos(0.0175*conj(q1) - 1.5708)*cos(0.0175*conj(q2) - 1.5708)*conj(q2d)*(conj(q3) + conj(L2)) + 0.0175*cos(0.0175*conj(q1) - 1.5708)*cos(0.0175*conj(q2) - 1.5708)*conj(q2d)*(conj(q3) + conj(L2)) + 0.0175*conj(q1d)*sin(0.0175*conj(q1) - 1.5708)*sin(0.0175*conj(q2) - 1.5708)*(conj(q3) + conj(L2)) - 0.0175*conj(q1d)*sin(0.0175*conj(q1) - 1.5708)*sin(0.0175*conj(q2) - 1.5708)*(conj(q3) + conj(L2)) - 0.0175*cos(0.0175*conj(q1) - 1.5708)*cos(0.0175*conj(q2) - 1.5708)*conj(q2d)*conj(L3) + 0.0175*cos(0.0175*conj(q1) - 1.5708)*cos(0.0175*conj(q2) - 1.5708)*conj(q2d)*conj(L3) + 0.0175*conj(q1d)*sin(0.0175*conj(q1) - 1.5708)*sin(0.0175*conj(q2) - 1.5708)*conj(L3) - 0.0175*conj(q1d)*sin(0.0175*conj(q1) - 1.5708)*sin(0.0175*conj(q2) - 1.5708)*conj(L3)) - (cos(0.0175*conj(q4) + 1.5708)*sin(0.0175*conj(q1) - 1.5708) + cos(0.0175*conj(q1) - 1.5708)*cos(0.0175*conj(q2) - 1.5708)*sin(0.0175*conj(q4) + 1.5708))*(cos(0.0175*conj(q2) - 1.5708)*conj(q3d) - cos(0.0175*conj(q2) - 1.5708)*conj(q3d) + conj(L4)*(0.0175*cos(0.0175*conj(q5) + 1.5708)*conj(q2d)*sin(0.0175*conj(q2) - 1.5708) + 0.0175*cos(0.0175*conj(q2) - 1.5708)*conj(q5d)*sin(0.0175*conj(q5) + 1.5708) - 0.0175*cos(0.0175*conj(q2) - 1.5708)*cos(0.0175*conj(q4) + 1.5708)*conj(q2d)*sin(0.0175*conj(q5) + 1.5708) - 0.0175*cos(0.0175*conj(q4) + 1.5708)*cos(0.0175*conj(q5) + 1.5708)*conj(q5d)*sin(0.0175*conj(q2) - 1.5708) + 0.0175*conj(q4d)*sin(0.0175*conj(q2) - 1.5708)*sin(0.0175*conj(q4) + 1.5708)*sin(0.0175*conj(q5) + 1.5708)) - 0.0175*conj(q2d)*sin(0.0175*conj(q2) - 1.5708)*conj(L3) + 0.0175*conj(q2d)*sin(0.0175*conj(q2) - 1.5708)*conj(L3) - 0.0175*conj(q2d)*sin(0.0175*conj(q2) - 1.5708)*(conj(q3) + conj(L2)) + 0.0175*conj(q2d)*sin(0.0175*conj(q2) - 1.5708)*(conj(q3) + conj(L2))) - (cos(0.0175*conj(q2) - 1.5708)*conj(L3) - cos(0.0175*conj(q2) - 1.5708)*conj(L3) + conj(L4)*(cos(0.0175*conj(q2) - 1.5708)*cos(0.0175*conj(q5) + 1.5708) + cos(0.0175*conj(q4) + 1.5708)*sin(0.0175*conj(q2) - 1.5708)*sin(0.0175*conj(q5) + 1.5708)) - cos(0.0175*conj(q2) - 1.5708)*(conj(q3) + conj(L2)) + cos(0.0175*conj(q2) - 1.5708)*(conj(q3) + conj(L2)))*(0.0175*conj(q4d)*sin(0.0175*conj(q1) - 1.5708)*sin(0.0175*conj(q4) + 1.5708) - 0.0175*cos(0.0175*conj(q1) - 1.5708)*cos(0.0175*conj(q4) + 1.5708)*conj(q1d) - 0.0175*cos(0.0175*conj(q1) - 1.5708)*cos(0.0175*conj(q2) - 1.5708)*cos(0.0175*conj(q4) + 1.5708)*conj(q4d) + 0.0175*cos(0.0175*conj(q2) - 1.5708)*conj(q1d)*sin(0.0175*conj(q1) - 1.5708)*sin(0.0175*conj(q4) + 1.5708) + 0.0175*cos(0.0175*conj(q1) - 1.5708)*conj(q2d)*sin(0.0175*conj(q2) - 1.5708)*sin(0.0175*conj(q4) + 1.5708)) + 0.0175*cos(0.0175*conj(q2) - 1.5708)*conj(q2d)*sin(0.0175*conj(q4) + 1.5708)*(conj(L4)*(sin(0.0175*conj(q5) + 1.5708)*(sin(0.0175*conj(q1) - 1.5708)*sin(0.0175*conj(q4) + 1.5708) - cos(0.0175*conj(q1) - 1.5708)*cos(0.0175*conj(q2) - 1.5708)*cos(0.0175*conj(q4) + 1.5708)) + cos(0.0175*conj(q1) - 1.5708)*cos(0.0175*conj(q5) + 1.5708)*sin(0.0175*conj(q2) - 1.5708)) - cos(0.0175*conj(q1) - 1.5708)*sin(0.0175*conj(q2) - 1.5708)*conj(L3) + cos(0.0175*conj(q1) - 1.5708)*sin(0.0175*conj(q2) - 1.5708)*conj(L3) - cos(0.0175*conj(q1) - 1.5708)*sin(0.0175*conj(q2) - 1.5708)*(conj(q3) + conj(L2)) + cos(0.0175*conj(q1) - 1.5708)*sin(0.0175*conj(q2) - 1.5708)*(conj(q3) + conj(L2))) + 0.0175*cos(0.0175*conj(q4) + 1.5708)*conj(q4d)*sin(0.0175*conj(q2) - 1.5708)*(conj(L4)*(sin(0.0175*conj(q5) + 1.5708)*(sin(0.0175*conj(q1) - 1.5708)*sin(0.0175*conj(q4) + 1.5708) - cos(0.0175*conj(q1) - 1.5708)*cos(0.0175*conj(q2) - 1.5708)*cos(0.0175*conj(q4) + 1.5708)) + cos(0.0175*conj(q1) - 1.5708)*cos(0.0175*conj(q5) + 1.5708)*sin(0.0175*conj(q2) - 1.5708)) - cos(0.0175*conj(q1) - 1.5708)*sin(0.0175*conj(q2) - 1.5708)*conj(L3) + cos(0.0175*conj(q1) - 1.5708)*sin(0.0175*conj(q2) - 1.5708)*conj(L3) - cos(0.0175*conj(q1) - 1.5708)*sin(0.0175*conj(q2) - 1.5708)*(conj(q3) + conj(L2)) + cos(0.0175*conj(q1) - 1.5708)*sin(0.0175*conj(q2) - 1.5708)*(conj(q3) + conj(L2))),                                                                                                                                                                                                                                                                                                                                                                                                                                                                                                                                                                                                                                                                                                                                                                                                                                                                                                                                                                                                                                                                                                                                                                                                                                                                                                                                                                                                                                                                                                                                                                                                                                                                                                                                                                                                                                                                                                                                                                                                                                                                                                                                                                                                                                                                                                                                                                                                                                                           (cos(0.0175*conj(q2) - 1.5708)*cos(0.0175*conj(q5) + 1.5708) + cos(0.0175*conj(q4) + 1.5708)*sin(0.0175*conj(q2) - 1.5708)*sin(0.0175*conj(q5) + 1.5708))*(conj(L4)*(sin(0.0175*conj(q5) + 1.5708)*(0.0175*cos(0.0175*conj(q1) - 1.5708)*conj(q1d)*sin(0.0175*conj(q4) + 1.5708) + 0.0175*cos(0.0175*conj(q4) + 1.5708)*conj(q4d)*sin(0.0175*conj(q1) - 1.5708) + 0.0175*cos(0.0175*conj(q2) - 1.5708)*cos(0.0175*conj(q4) + 1.5708)*conj(q1d)*sin(0.0175*conj(q1) - 1.5708) + 0.0175*cos(0.0175*conj(q1) - 1.5708)*cos(0.0175*conj(q4) + 1.5708)*conj(q2d)*sin(0.0175*conj(q2) - 1.5708) + 0.0175*cos(0.0175*conj(q1) - 1.5708)*cos(0.0175*conj(q2) - 1.5708)*conj(q4d)*sin(0.0175*conj(q4) + 1.5708)) + 0.0175*cos(0.0175*conj(q5) + 1.5708)*conj(q5d)*(sin(0.0175*conj(q1) - 1.5708)*sin(0.0175*conj(q4) + 1.5708) - cos(0.0175*conj(q1) - 1.5708)*cos(0.0175*conj(q2) - 1.5708)*cos(0.0175*conj(q4) + 1.5708)) + 0.0175*cos(0.0175*conj(q1) - 1.5708)*cos(0.0175*conj(q2) - 1.5708)*cos(0.0175*conj(q5) + 1.5708)*conj(q2d) - 0.0175*cos(0.0175*conj(q5) + 1.5708)*conj(q1d)*sin(0.0175*conj(q1) - 1.5708)*sin(0.0175*conj(q2) - 1.5708) - 0.0175*cos(0.0175*conj(q1) - 1.5708)*conj(q5d)*sin(0.0175*conj(q2) - 1.5708)*sin(0.0175*conj(q5) + 1.5708)) - cos(0.0175*conj(q1) - 1.5708)*conj(q3d)*sin(0.0175*conj(q2) - 1.5708) + cos(0.0175*conj(q1) - 1.5708)*conj(q3d)*sin(0.0175*conj(q2) - 1.5708) - 0.0175*cos(0.0175*conj(q1) - 1.5708)*cos(0.0175*conj(q2) - 1.5708)*conj(q2d)*(conj(q3) + conj(L2)) + 0.0175*cos(0.0175*conj(q1) - 1.5708)*cos(0.0175*conj(q2) - 1.5708)*conj(q2d)*(conj(q3) + conj(L2)) + 0.0175*conj(q1d)*sin(0.0175*conj(q1) - 1.5708)*sin(0.0175*conj(q2) - 1.5708)*(conj(q3) + conj(L2)) - 0.0175*conj(q1d)*sin(0.0175*conj(q1) - 1.5708)*sin(0.0175*conj(q2) - 1.5708)*(conj(q3) + conj(L2)) - 0.0175*cos(0.0175*conj(q1) - 1.5708)*cos(0.0175*conj(q2) - 1.5708)*conj(q2d)*conj(L3) + 0.0175*cos(0.0175*conj(q1) - 1.5708)*cos(0.0175*conj(q2) - 1.5708)*conj(q2d)*conj(L3) + 0.0175*conj(q1d)*sin(0.0175*conj(q1) - 1.5708)*sin(0.0175*conj(q2) - 1.5708)*conj(L3) - 0.0175*conj(q1d)*sin(0.0175*conj(q1) - 1.5708)*sin(0.0175*conj(q2) - 1.5708)*conj(L3)) - (conj(L4)*(sin(0.0175*conj(q5) + 1.5708)*(sin(0.0175*conj(q1) - 1.5708)*sin(0.0175*conj(q4) + 1.5708) - cos(0.0175*conj(q1) - 1.5708)*cos(0.0175*conj(q2) - 1.5708)*cos(0.0175*conj(q4) + 1.5708)) + cos(0.0175*conj(q1) - 1.5708)*cos(0.0175*conj(q5) + 1.5708)*sin(0.0175*conj(q2) - 1.5708)) - cos(0.0175*conj(q1) - 1.5708)*sin(0.0175*conj(q2) - 1.5708)*conj(L3) + cos(0.0175*conj(q1) - 1.5708)*sin(0.0175*conj(q2) - 1.5708)*conj(L3) - cos(0.0175*conj(q1) - 1.5708)*sin(0.0175*conj(q2) - 1.5708)*(conj(q3) + conj(L2)) + cos(0.0175*conj(q1) - 1.5708)*sin(0.0175*conj(q2) - 1.5708)*(conj(q3) + conj(L2)))*(0.0175*cos(0.0175*conj(q5) + 1.5708)*conj(q2d)*sin(0.0175*conj(q2) - 1.5708) + 0.0175*cos(0.0175*conj(q2) - 1.5708)*conj(q5d)*sin(0.0175*conj(q5) + 1.5708) - 0.0175*cos(0.0175*conj(q2) - 1.5708)*cos(0.0175*conj(q4) + 1.5708)*conj(q2d)*sin(0.0175*conj(q5) + 1.5708) - 0.0175*cos(0.0175*conj(q4) + 1.5708)*cos(0.0175*conj(q5) + 1.5708)*conj(q5d)*sin(0.0175*conj(q2) - 1.5708) + 0.0175*conj(q4d)*sin(0.0175*conj(q2) - 1.5708)*sin(0.0175*conj(q4) + 1.5708)*sin(0.0175*conj(q5) + 1.5708)) - (cos(0.0175*conj(q2) - 1.5708)*conj(L3) - cos(0.0175*conj(q2) - 1.5708)*conj(L3) + conj(L4)*(cos(0.0175*conj(q2) - 1.5708)*cos(0.0175*conj(q5) + 1.5708) + cos(0.0175*conj(q4) + 1.5708)*sin(0.0175*conj(q2) - 1.5708)*sin(0.0175*conj(q5) + 1.5708)) - cos(0.0175*conj(q2) - 1.5708)*(conj(q3) + conj(L2)) + cos(0.0175*conj(q2) - 1.5708)*(conj(q3) + conj(L2)))*(sin(0.0175*conj(q5) + 1.5708)*(0.0175*cos(0.0175*conj(q1) - 1.5708)*conj(q1d)*sin(0.0175*conj(q4) + 1.5708) + 0.0175*cos(0.0175*conj(q4) + 1.5708)*conj(q4d)*sin(0.0175*conj(q1) - 1.5708) + 0.0175*cos(0.0175*conj(q2) - 1.5708)*cos(0.0175*conj(q4) + 1.5708)*conj(q1d)*sin(0.0175*conj(q1) - 1.5708) + 0.0175*cos(0.0175*conj(q1) - 1.5708)*cos(0.0175*conj(q4) + 1.5708)*conj(q2d)*sin(0.0175*conj(q2) - 1.5708) + 0.0175*cos(0.0175*conj(q1) - 1.5708)*cos(0.0175*conj(q2) - 1.5708)*conj(q4d)*sin(0.0175*conj(q4) + 1.5708)) + 0.0175*cos(0.0175*conj(q5) + 1.5708)*conj(q5d)*(sin(0.0175*conj(q1) - 1.5708)*sin(0.0175*conj(q4) + 1.5708) - cos(0.0175*conj(q1) - 1.5708)*cos(0.0175*conj(q2) - 1.5708)*cos(0.0175*conj(q4) + 1.5708)) + 0.0175*cos(0.0175*conj(q1) - 1.5708)*cos(0.0175*conj(q2) - 1.5708)*cos(0.0175*conj(q5) + 1.5708)*conj(q2d) - 0.0175*cos(0.0175*conj(q5) + 1.5708)*conj(q1d)*sin(0.0175*conj(q1) - 1.5708)*sin(0.0175*conj(q2) - 1.5708) - 0.0175*cos(0.0175*conj(q1) - 1.5708)*conj(q5d)*sin(0.0175*conj(q2) - 1.5708)*sin(0.0175*conj(q5) + 1.5708)) + (sin(0.0175*conj(q5) + 1.5708)*(sin(0.0175*conj(q1) - 1.5708)*sin(0.0175*conj(q4) + 1.5708) - cos(0.0175*conj(q1) - 1.5708)*cos(0.0175*conj(q2) - 1.5708)*cos(0.0175*conj(q4) + 1.5708)) + cos(0.0175*conj(q1) - 1.5708)*cos(0.0175*conj(q5) + 1.5708)*sin(0.0175*conj(q2) - 1.5708))*(cos(0.0175*conj(q2) - 1.5708)*conj(q3d) - cos(0.0175*conj(q2) - 1.5708)*conj(q3d) + conj(L4)*(0.0175*cos(0.0175*conj(q5) + 1.5708)*conj(q2d)*sin(0.0175*conj(q2) - 1.5708) + 0.0175*cos(0.0175*conj(q2) - 1.5708)*conj(q5d)*sin(0.0175*conj(q5) + 1.5708) - 0.0175*cos(0.0175*conj(q2) - 1.5708)*cos(0.0175*conj(q4) + 1.5708)*conj(q2d)*sin(0.0175*conj(q5) + 1.5708) - 0.0175*cos(0.0175*conj(q4) + 1.5708)*cos(0.0175*conj(q5) + 1.5708)*conj(q5d)*sin(0.0175*conj(q2) - 1.5708) + 0.0175*conj(q4d)*sin(0.0175*conj(q2) - 1.5708)*sin(0.0175*conj(q4) + 1.5708)*sin(0.0175*conj(q5) + 1.5708)) - 0.0175*conj(q2d)*sin(0.0175*conj(q2) - 1.5708)*conj(L3) + 0.0175*conj(q2d)*sin(0.0175*conj(q2) - 1.5708)*conj(L3) - 0.0175*conj(q2d)*sin(0.0175*conj(q2) - 1.5708)*(conj(q3) + conj(L2)) + 0.0175*conj(q2d)*sin(0.0175*conj(q2) - 1.5708)*(conj(q3) + conj(L2)));
                                                                                                                                                                                                                                                                                                                                                                                                                                                                                                                                                                                                                                                                                                                                                                                                                                                                                                                                                                                                                                                                                                                                                                                                                                                                                                                                                                                                                                                                                                                                                                                                                                                                                                                                                                                                                                                      0, cos(0.0175*conj(q1) - 1.5708)*(conj(L4)*(sin(0.0175*conj(q5) + 1.5708)*(0.0175*cos(0.0175*conj(q1) - 1.5708)*conj(q1d)*sin(0.0175*conj(q4) + 1.5708) + 0.0175*cos(0.0175*conj(q4) + 1.5708)*conj(q4d)*sin(0.0175*conj(q1) - 1.5708) + 0.0175*cos(0.0175*conj(q2) - 1.5708)*cos(0.0175*conj(q4) + 1.5708)*conj(q1d)*sin(0.0175*conj(q1) - 1.5708) + 0.0175*cos(0.0175*conj(q1) - 1.5708)*cos(0.0175*conj(q4) + 1.5708)*conj(q2d)*sin(0.0175*conj(q2) - 1.5708) + 0.0175*cos(0.0175*conj(q1) - 1.5708)*cos(0.0175*conj(q2) - 1.5708)*conj(q4d)*sin(0.0175*conj(q4) + 1.5708)) + 0.0175*cos(0.0175*conj(q5) + 1.5708)*conj(q5d)*(sin(0.0175*conj(q1) - 1.5708)*sin(0.0175*conj(q4) + 1.5708) - cos(0.0175*conj(q1) - 1.5708)*cos(0.0175*conj(q2) - 1.5708)*cos(0.0175*conj(q4) + 1.5708)) + 0.0175*cos(0.0175*conj(q1) - 1.5708)*cos(0.0175*conj(q2) - 1.5708)*cos(0.0175*conj(q5) + 1.5708)*conj(q2d) - 0.0175*cos(0.0175*conj(q5) + 1.5708)*conj(q1d)*sin(0.0175*conj(q1) - 1.5708)*sin(0.0175*conj(q2) - 1.5708) - 0.0175*cos(0.0175*conj(q1) - 1.5708)*conj(q5d)*sin(0.0175*conj(q2) - 1.5708)*sin(0.0175*conj(q5) + 1.5708)) - cos(0.0175*conj(q1) - 1.5708)*conj(q3d)*sin(0.0175*conj(q2) - 1.5708) - 0.0175*cos(0.0175*conj(q1) - 1.5708)*cos(0.0175*conj(q2) - 1.5708)*conj(q2d)*(conj(q3) + conj(L2)) + 0.0175*conj(q1d)*sin(0.0175*conj(q1) - 1.5708)*sin(0.0175*conj(q2) - 1.5708)*(conj(q3) + conj(L2)) - 0.0175*cos(0.0175*conj(q1) - 1.5708)*cos(0.0175*conj(q2) - 1.5708)*conj(q2d)*conj(L3) + 0.0175*conj(q1d)*sin(0.0175*conj(q1) - 1.5708)*sin(0.0175*conj(q2) - 1.5708)*conj(L3)) - sin(0.0175*conj(q1) - 1.5708)*(conj(q3d)*sin(0.0175*conj(q1) - 1.5708)*sin(0.0175*conj(q2) - 1.5708) - conj(L4)*(sin(0.0175*conj(q5) + 1.5708)*(0.0175*conj(q1d)*sin(0.0175*conj(q1) - 1.5708)*sin(0.0175*conj(q4) + 1.5708) - 0.0175*cos(0.0175*conj(q1) - 1.5708)*cos(0.0175*conj(q4) + 1.5708)*conj(q4d) - 0.0175*cos(0.0175*conj(q1) - 1.5708)*cos(0.0175*conj(q2) - 1.5708)*cos(0.0175*conj(q4) + 1.5708)*conj(q1d) + 0.0175*cos(0.0175*conj(q4) + 1.5708)*conj(q2d)*sin(0.0175*conj(q1) - 1.5708)*sin(0.0175*conj(q2) - 1.5708) + 0.0175*cos(0.0175*conj(q2) - 1.5708)*conj(q4d)*sin(0.0175*conj(q1) - 1.5708)*sin(0.0175*conj(q4) + 1.5708)) - 0.0175*cos(0.0175*conj(q5) + 1.5708)*conj(q5d)*(cos(0.0175*conj(q1) - 1.5708)*sin(0.0175*conj(q4) + 1.5708) + cos(0.0175*conj(q2) - 1.5708)*cos(0.0175*conj(q4) + 1.5708)*sin(0.0175*conj(q1) - 1.5708)) + 0.0175*cos(0.0175*conj(q1) - 1.5708)*cos(0.0175*conj(q5) + 1.5708)*conj(q1d)*sin(0.0175*conj(q2) - 1.5708) + 0.0175*cos(0.0175*conj(q2) - 1.5708)*cos(0.0175*conj(q5) + 1.5708)*conj(q2d)*sin(0.0175*conj(q1) - 1.5708) - 0.0175*conj(q5d)*sin(0.0175*conj(q1) - 1.5708)*sin(0.0175*conj(q2) - 1.5708)*sin(0.0175*conj(q5) + 1.5708)) + 0.0175*cos(0.0175*conj(q1) - 1.5708)*conj(q1d)*sin(0.0175*conj(q2) - 1.5708)*(conj(q3) + conj(L2)) + 0.0175*cos(0.0175*conj(q2) - 1.5708)*conj(q2d)*sin(0.0175*conj(q1) - 1.5708)*(conj(q3) + conj(L2)) + 0.0175*cos(0.0175*conj(q1) - 1.5708)*conj(q1d)*sin(0.0175*conj(q2) - 1.5708)*conj(L3) + 0.0175*cos(0.0175*conj(q2) - 1.5708)*conj(q2d)*sin(0.0175*conj(q1) - 1.5708)*conj(L3)) + 0.0175*conj(q1d)*sin(0.0175*conj(q1) - 1.5708)*(cos(0.0175*conj(q1) - 1.5708)*sin(0.0175*conj(q2) - 1.5708)*conj(L3) - conj(L4)*(sin(0.0175*conj(q5) + 1.5708)*(sin(0.0175*conj(q1) - 1.5708)*sin(0.0175*conj(q4) + 1.5708) - cos(0.0175*conj(q1) - 1.5708)*cos(0.0175*conj(q2) - 1.5708)*cos(0.0175*conj(q4) + 1.5708)) + cos(0.0175*conj(q1) - 1.5708)*cos(0.0175*conj(q5) + 1.5708)*sin(0.0175*conj(q2) - 1.5708)) + cos(0.0175*conj(q1) - 1.5708)*sin(0.0175*conj(q2) - 1.5708)*(conj(q3) + conj(L2))) - 0.0175*cos(0.0175*conj(q1) - 1.5708)*conj(q1d)*(conj(L4)*(sin(0.0175*conj(q5) + 1.5708)*(cos(0.0175*conj(q1) - 1.5708)*sin(0.0175*conj(q4) + 1.5708) + cos(0.0175*conj(q2) - 1.5708)*cos(0.0175*conj(q4) + 1.5708)*sin(0.0175*conj(q1) - 1.5708)) - cos(0.0175*conj(q5) + 1.5708)*sin(0.0175*conj(q1) - 1.5708)*sin(0.0175*conj(q2) - 1.5708)) + sin(0.0175*conj(q1) - 1.5708)*sin(0.0175*conj(q2) - 1.5708)*(conj(q3) + conj(L2)) + sin(0.0175*conj(q1) - 1.5708)*sin(0.0175*conj(q2) - 1.5708)*conj(L3)),                                                                                                         -0.0175*sin(0.0175*q2 - 1.5708)*q2d, sin(0.0175*conj(q1) - 1.5708)*sin(0.0175*conj(q2) - 1.5708)*(conj(L4)*(sin(0.0175*conj(q5) + 1.5708)*(0.0175*cos(0.0175*conj(q1) - 1.5708)*conj(q1d)*sin(0.0175*conj(q4) + 1.5708) + 0.0175*cos(0.0175*conj(q4) + 1.5708)*conj(q4d)*sin(0.0175*conj(q1) - 1.5708) + 0.0175*cos(0.0175*conj(q2) - 1.5708)*cos(0.0175*conj(q4) + 1.5708)*conj(q1d)*sin(0.0175*conj(q1) - 1.5708) + 0.0175*cos(0.0175*conj(q1) - 1.5708)*cos(0.0175*conj(q4) + 1.5708)*conj(q2d)*sin(0.0175*conj(q2) - 1.5708) + 0.0175*cos(0.0175*conj(q1) - 1.5708)*cos(0.0175*conj(q2) - 1.5708)*conj(q4d)*sin(0.0175*conj(q4) + 1.5708)) + 0.0175*cos(0.0175*conj(q5) + 1.5708)*conj(q5d)*(sin(0.0175*conj(q1) - 1.5708)*sin(0.0175*conj(q4) + 1.5708) - cos(0.0175*conj(q1) - 1.5708)*cos(0.0175*conj(q2) - 1.5708)*cos(0.0175*conj(q4) + 1.5708)) + 0.0175*cos(0.0175*conj(q1) - 1.5708)*cos(0.0175*conj(q2) - 1.5708)*cos(0.0175*conj(q5) + 1.5708)*conj(q2d) - 0.0175*cos(0.0175*conj(q5) + 1.5708)*conj(q1d)*sin(0.0175*conj(q1) - 1.5708)*sin(0.0175*conj(q2) - 1.5708) - 0.0175*cos(0.0175*conj(q1) - 1.5708)*conj(q5d)*sin(0.0175*conj(q2) - 1.5708)*sin(0.0175*conj(q5) + 1.5708)) - cos(0.0175*conj(q1) - 1.5708)*conj(q3d)*sin(0.0175*conj(q2) - 1.5708) + cos(0.0175*conj(q1) - 1.5708)*conj(q3d)*sin(0.0175*conj(q2) - 1.5708) - 0.0175*cos(0.0175*conj(q1) - 1.5708)*cos(0.0175*conj(q2) - 1.5708)*conj(q2d)*(conj(q3) + conj(L2)) + 0.0175*cos(0.0175*conj(q1) - 1.5708)*cos(0.0175*conj(q2) - 1.5708)*conj(q2d)*(conj(q3) + conj(L2)) + 0.0175*conj(q1d)*sin(0.0175*conj(q1) - 1.5708)*sin(0.0175*conj(q2) - 1.5708)*(conj(q3) + conj(L2)) - 0.0175*conj(q1d)*sin(0.0175*conj(q1) - 1.5708)*sin(0.0175*conj(q2) - 1.5708)*(conj(q3) + conj(L2)) - 0.0175*cos(0.0175*conj(q1) - 1.5708)*cos(0.0175*conj(q2) - 1.5708)*conj(q2d)*conj(L3) + 0.0175*conj(q1d)*sin(0.0175*conj(q1) - 1.5708)*sin(0.0175*conj(q2) - 1.5708)*conj(L3)) + cos(0.0175*conj(q1) - 1.5708)*sin(0.0175*conj(q2) - 1.5708)*(conj(q3d)*sin(0.0175*conj(q1) - 1.5708)*sin(0.0175*conj(q2) - 1.5708) - conj(L4)*(sin(0.0175*conj(q5) + 1.5708)*(0.0175*conj(q1d)*sin(0.0175*conj(q1) - 1.5708)*sin(0.0175*conj(q4) + 1.5708) - 0.0175*cos(0.0175*conj(q1) - 1.5708)*cos(0.0175*conj(q4) + 1.5708)*conj(q4d) - 0.0175*cos(0.0175*conj(q1) - 1.5708)*cos(0.0175*conj(q2) - 1.5708)*cos(0.0175*conj(q4) + 1.5708)*conj(q1d) + 0.0175*cos(0.0175*conj(q4) + 1.5708)*conj(q2d)*sin(0.0175*conj(q1) - 1.5708)*sin(0.0175*conj(q2) - 1.5708) + 0.0175*cos(0.0175*conj(q2) - 1.5708)*conj(q4d)*sin(0.0175*conj(q1) - 1.5708)*sin(0.0175*conj(q4) + 1.5708)) - 0.0175*cos(0.0175*conj(q5) + 1.5708)*conj(q5d)*(cos(0.0175*conj(q1) - 1.5708)*sin(0.0175*conj(q4) + 1.5708) + cos(0.0175*conj(q2) - 1.5708)*cos(0.0175*conj(q4) + 1.5708)*sin(0.0175*conj(q1) - 1.5708)) + 0.0175*cos(0.0175*conj(q1) - 1.5708)*cos(0.0175*conj(q5) + 1.5708)*conj(q1d)*sin(0.0175*conj(q2) - 1.5708) + 0.0175*cos(0.0175*conj(q2) - 1.5708)*cos(0.0175*conj(q5) + 1.5708)*conj(q2d)*sin(0.0175*conj(q1) - 1.5708) - 0.0175*conj(q5d)*sin(0.0175*conj(q1) - 1.5708)*sin(0.0175*conj(q2) - 1.5708)*sin(0.0175*conj(q5) + 1.5708)) - conj(q3d)*sin(0.0175*conj(q1) - 1.5708)*sin(0.0175*conj(q2) - 1.5708) + 0.0175*cos(0.0175*conj(q1) - 1.5708)*conj(q1d)*sin(0.0175*conj(q2) - 1.5708)*(conj(q3) + conj(L2)) + 0.0175*cos(0.0175*conj(q2) - 1.5708)*conj(q2d)*sin(0.0175*conj(q1) - 1.5708)*(conj(q3) + conj(L2)) - 0.0175*cos(0.0175*conj(q1) - 1.5708)*conj(q1d)*sin(0.0175*conj(q2) - 1.5708)*(conj(q3) + conj(L2)) - 0.0175*cos(0.0175*conj(q2) - 1.5708)*conj(q2d)*sin(0.0175*conj(q1) - 1.5708)*(conj(q3) + conj(L2)) + 0.0175*cos(0.0175*conj(q1) - 1.5708)*conj(q1d)*sin(0.0175*conj(q2) - 1.5708)*conj(L3) + 0.0175*cos(0.0175*conj(q2) - 1.5708)*conj(q2d)*sin(0.0175*conj(q1) - 1.5708)*conj(L3)) + 0.0175*cos(0.0175*conj(q1) - 1.5708)*conj(q1d)*sin(0.0175*conj(q2) - 1.5708)*(conj(L4)*(sin(0.0175*conj(q5) + 1.5708)*(sin(0.0175*conj(q1) - 1.5708)*sin(0.0175*conj(q4) + 1.5708) - cos(0.0175*conj(q1) - 1.5708)*cos(0.0175*conj(q2) - 1.5708)*cos(0.0175*conj(q4) + 1.5708)) + cos(0.0175*conj(q1) - 1.5708)*cos(0.0175*conj(q5) + 1.5708)*sin(0.0175*conj(q2) - 1.5708)) - cos(0.0175*conj(q1) - 1.5708)*sin(0.0175*conj(q2) - 1.5708)*conj(L3) - cos(0.0175*conj(q1) - 1.5708)*sin(0.0175*conj(q2) - 1.5708)*(conj(q3) + conj(L2)) + cos(0.0175*conj(q1) - 1.5708)*sin(0.0175*conj(q2) - 1.5708)*(conj(q3) + conj(L2))) + 0.0175*cos(0.0175*conj(q2) - 1.5708)*conj(q2d)*sin(0.0175*conj(q1) - 1.5708)*(conj(L4)*(sin(0.0175*conj(q5) + 1.5708)*(sin(0.0175*conj(q1) - 1.5708)*sin(0.0175*conj(q4) + 1.5708) - cos(0.0175*conj(q1) - 1.5708)*cos(0.0175*conj(q2) - 1.5708)*cos(0.0175*conj(q4) + 1.5708)) + cos(0.0175*conj(q1) - 1.5708)*cos(0.0175*conj(q5) + 1.5708)*sin(0.0175*conj(q2) - 1.5708)) - cos(0.0175*conj(q1) - 1.5708)*sin(0.0175*conj(q2) - 1.5708)*conj(L3) - cos(0.0175*conj(q1) - 1.5708)*sin(0.0175*conj(q2) - 1.5708)*(conj(q3) + conj(L2)) + cos(0.0175*conj(q1) - 1.5708)*sin(0.0175*conj(q2) - 1.5708)*(conj(q3) + conj(L2))) + 0.0175*cos(0.0175*conj(q1) - 1.5708)*cos(0.0175*conj(q2) - 1.5708)*conj(q2d)*(conj(L4)*(sin(0.0175*conj(q5) + 1.5708)*(cos(0.0175*conj(q1) - 1.5708)*sin(0.0175*conj(q4) + 1.5708) + cos(0.0175*conj(q2) - 1.5708)*cos(0.0175*conj(q4) + 1.5708)*sin(0.0175*conj(q1) - 1.5708)) - cos(0.0175*conj(q5) + 1.5708)*sin(0.0175*conj(q1) - 1.5708)*sin(0.0175*conj(q2) - 1.5708)) + sin(0.0175*conj(q1) - 1.5708)*sin(0.0175*conj(q2) - 1.5708)*(conj(q3) + conj(L2)) - sin(0.0175*conj(q1) - 1.5708)*sin(0.0175*conj(q2) - 1.5708)*(conj(q3) + conj(L2)) + sin(0.0175*conj(q1) - 1.5708)*sin(0.0175*conj(q2) - 1.5708)*conj(L3)) - 0.0175*conj(q1d)*sin(0.0175*conj(q1) - 1.5708)*sin(0.0175*conj(q2) - 1.5708)*(conj(L4)*(sin(0.0175*conj(q5) + 1.5708)*(cos(0.0175*conj(q1) - 1.5708)*sin(0.0175*conj(q4) + 1.5708) + cos(0.0175*conj(q2) - 1.5708)*cos(0.0175*conj(q4) + 1.5708)*sin(0.0175*conj(q1) - 1.5708)) - cos(0.0175*conj(q5) + 1.5708)*sin(0.0175*conj(q1) - 1.5708)*sin(0.0175*conj(q2) - 1.5708)) + sin(0.0175*conj(q1) - 1.5708)*sin(0.0175*conj(q2) - 1.5708)*(conj(q3) + conj(L2)) - sin(0.0175*conj(q1) - 1.5708)*sin(0.0175*conj(q2) - 1.5708)*(conj(q3) + conj(L2)) + sin(0.0175*conj(q1) - 1.5708)*sin(0.0175*conj(q2) - 1.5708)*conj(L3)), (conj(L4)*(sin(0.0175*conj(q5) + 1.5708)*(sin(0.0175*conj(q1) - 1.5708)*sin(0.0175*conj(q4) + 1.5708) - cos(0.0175*conj(q1) - 1.5708)*cos(0.0175*conj(q2) - 1.5708)*cos(0.0175*conj(q4) + 1.5708)) + cos(0.0175*conj(q1) - 1.5708)*cos(0.0175*conj(q5) + 1.5708)*sin(0.0175*conj(q2) - 1.5708)) - cos(0.0175*conj(q1) - 1.5708)*sin(0.0175*conj(q2) - 1.5708)*conj(L3) + cos(0.0175*conj(q1) - 1.5708)*sin(0.0175*conj(q2) - 1.5708)*conj(L3) - cos(0.0175*conj(q1) - 1.5708)*sin(0.0175*conj(q2) - 1.5708)*(conj(q3) + conj(L2)) + cos(0.0175*conj(q1) - 1.5708)*sin(0.0175*conj(q2) - 1.5708)*(conj(q3) + conj(L2)))*(0.0175*cos(0.0175*conj(q4) + 1.5708)*conj(q1d)*sin(0.0175*conj(q1) - 1.5708) + 0.0175*cos(0.0175*conj(q1) - 1.5708)*conj(q4d)*sin(0.0175*conj(q4) + 1.5708) + 0.0175*cos(0.0175*conj(q1) - 1.5708)*cos(0.0175*conj(q2) - 1.5708)*conj(q1d)*sin(0.0175*conj(q4) + 1.5708) + 0.0175*cos(0.0175*conj(q2) - 1.5708)*cos(0.0175*conj(q4) + 1.5708)*conj(q4d)*sin(0.0175*conj(q1) - 1.5708) - 0.0175*conj(q2d)*sin(0.0175*conj(q1) - 1.5708)*sin(0.0175*conj(q2) - 1.5708)*sin(0.0175*conj(q4) + 1.5708)) - (cos(0.0175*conj(q4) + 1.5708)*sin(0.0175*conj(q1) - 1.5708) + cos(0.0175*conj(q1) - 1.5708)*cos(0.0175*conj(q2) - 1.5708)*sin(0.0175*conj(q4) + 1.5708))*(conj(L4)*(sin(0.0175*conj(q5) + 1.5708)*(0.0175*conj(q1d)*sin(0.0175*conj(q1) - 1.5708)*sin(0.0175*conj(q4) + 1.5708) - 0.0175*cos(0.0175*conj(q1) - 1.5708)*cos(0.0175*conj(q4) + 1.5708)*conj(q4d) - 0.0175*cos(0.0175*conj(q1) - 1.5708)*cos(0.0175*conj(q2) - 1.5708)*cos(0.0175*conj(q4) + 1.5708)*conj(q1d) + 0.0175*cos(0.0175*conj(q4) + 1.5708)*conj(q2d)*sin(0.0175*conj(q1) - 1.5708)*sin(0.0175*conj(q2) - 1.5708) + 0.0175*cos(0.0175*conj(q2) - 1.5708)*conj(q4d)*sin(0.0175*conj(q1) - 1.5708)*sin(0.0175*conj(q4) + 1.5708)) - 0.0175*cos(0.0175*conj(q5) + 1.5708)*conj(q5d)*(cos(0.0175*conj(q1) - 1.5708)*sin(0.0175*conj(q4) + 1.5708) + cos(0.0175*conj(q2) - 1.5708)*cos(0.0175*conj(q4) + 1.5708)*sin(0.0175*conj(q1) - 1.5708)) + 0.0175*cos(0.0175*conj(q1) - 1.5708)*cos(0.0175*conj(q5) + 1.5708)*conj(q1d)*sin(0.0175*conj(q2) - 1.5708) + 0.0175*cos(0.0175*conj(q2) - 1.5708)*cos(0.0175*conj(q5) + 1.5708)*conj(q2d)*sin(0.0175*conj(q1) - 1.5708) - 0.0175*conj(q5d)*sin(0.0175*conj(q1) - 1.5708)*sin(0.0175*conj(q2) - 1.5708)*sin(0.0175*conj(q5) + 1.5708)) - conj(q3d)*sin(0.0175*conj(q1) - 1.5708)*sin(0.0175*conj(q2) - 1.5708) + conj(q3d)*sin(0.0175*conj(q1) - 1.5708)*sin(0.0175*conj(q2) - 1.5708) - 0.0175*cos(0.0175*conj(q1) - 1.5708)*conj(q1d)*sin(0.0175*conj(q2) - 1.5708)*(conj(q3) + conj(L2)) - 0.0175*cos(0.0175*conj(q2) - 1.5708)*conj(q2d)*sin(0.0175*conj(q1) - 1.5708)*(conj(q3) + conj(L2)) + 0.0175*cos(0.0175*conj(q1) - 1.5708)*conj(q1d)*sin(0.0175*conj(q2) - 1.5708)*(conj(q3) + conj(L2)) + 0.0175*cos(0.0175*conj(q2) - 1.5708)*conj(q2d)*sin(0.0175*conj(q1) - 1.5708)*(conj(q3) + conj(L2)) - 0.0175*cos(0.0175*conj(q1) - 1.5708)*conj(q1d)*sin(0.0175*conj(q2) - 1.5708)*conj(L3) - 0.0175*cos(0.0175*conj(q2) - 1.5708)*conj(q2d)*sin(0.0175*conj(q1) - 1.5708)*conj(L3) + 0.0175*cos(0.0175*conj(q1) - 1.5708)*conj(q1d)*sin(0.0175*conj(q2) - 1.5708)*conj(L3) + 0.0175*cos(0.0175*conj(q2) - 1.5708)*conj(q2d)*sin(0.0175*conj(q1) - 1.5708)*conj(L3)) - (conj(L4)*(sin(0.0175*conj(q5) + 1.5708)*(cos(0.0175*conj(q1) - 1.5708)*sin(0.0175*conj(q4) + 1.5708) + cos(0.0175*conj(q2) - 1.5708)*cos(0.0175*conj(q4) + 1.5708)*sin(0.0175*conj(q1) - 1.5708)) - cos(0.0175*conj(q5) + 1.5708)*sin(0.0175*conj(q1) - 1.5708)*sin(0.0175*conj(q2) - 1.5708)) + sin(0.0175*conj(q1) - 1.5708)*sin(0.0175*conj(q2) - 1.5708)*(conj(q3) + conj(L2)) - sin(0.0175*conj(q1) - 1.5708)*sin(0.0175*conj(q2) - 1.5708)*(conj(q3) + conj(L2)) + sin(0.0175*conj(q1) - 1.5708)*sin(0.0175*conj(q2) - 1.5708)*conj(L3) - sin(0.0175*conj(q1) - 1.5708)*sin(0.0175*conj(q2) - 1.5708)*conj(L3))*(0.0175*conj(q4d)*sin(0.0175*conj(q1) - 1.5708)*sin(0.0175*conj(q4) + 1.5708) - 0.0175*cos(0.0175*conj(q1) - 1.5708)*cos(0.0175*conj(q4) + 1.5708)*conj(q1d) - 0.0175*cos(0.0175*conj(q1) - 1.5708)*cos(0.0175*conj(q2) - 1.5708)*cos(0.0175*conj(q4) + 1.5708)*conj(q4d) + 0.0175*cos(0.0175*conj(q2) - 1.5708)*conj(q1d)*sin(0.0175*conj(q1) - 1.5708)*sin(0.0175*conj(q4) + 1.5708) + 0.0175*cos(0.0175*conj(q1) - 1.5708)*conj(q2d)*sin(0.0175*conj(q2) - 1.5708)*sin(0.0175*conj(q4) + 1.5708)) - (cos(0.0175*conj(q1) - 1.5708)*cos(0.0175*conj(q4) + 1.5708) - cos(0.0175*conj(q2) - 1.5708)*sin(0.0175*conj(q1) - 1.5708)*sin(0.0175*conj(q4) + 1.5708))*(conj(L4)*(sin(0.0175*conj(q5) + 1.5708)*(0.0175*cos(0.0175*conj(q1) - 1.5708)*conj(q1d)*sin(0.0175*conj(q4) + 1.5708) + 0.0175*cos(0.0175*conj(q4) + 1.5708)*conj(q4d)*sin(0.0175*conj(q1) - 1.5708) + 0.0175*cos(0.0175*conj(q2) - 1.5708)*cos(0.0175*conj(q4) + 1.5708)*conj(q1d)*sin(0.0175*conj(q1) - 1.5708) + 0.0175*cos(0.0175*conj(q1) - 1.5708)*cos(0.0175*conj(q4) + 1.5708)*conj(q2d)*sin(0.0175*conj(q2) - 1.5708) + 0.0175*cos(0.0175*conj(q1) - 1.5708)*cos(0.0175*conj(q2) - 1.5708)*conj(q4d)*sin(0.0175*conj(q4) + 1.5708)) + 0.0175*cos(0.0175*conj(q5) + 1.5708)*conj(q5d)*(sin(0.0175*conj(q1) - 1.5708)*sin(0.0175*conj(q4) + 1.5708) - cos(0.0175*conj(q1) - 1.5708)*cos(0.0175*conj(q2) - 1.5708)*cos(0.0175*conj(q4) + 1.5708)) + 0.0175*cos(0.0175*conj(q1) - 1.5708)*cos(0.0175*conj(q2) - 1.5708)*cos(0.0175*conj(q5) + 1.5708)*conj(q2d) - 0.0175*cos(0.0175*conj(q5) + 1.5708)*conj(q1d)*sin(0.0175*conj(q1) - 1.5708)*sin(0.0175*conj(q2) - 1.5708) - 0.0175*cos(0.0175*conj(q1) - 1.5708)*conj(q5d)*sin(0.0175*conj(q2) - 1.5708)*sin(0.0175*conj(q5) + 1.5708)) - cos(0.0175*conj(q1) - 1.5708)*conj(q3d)*sin(0.0175*conj(q2) - 1.5708) + cos(0.0175*conj(q1) - 1.5708)*conj(q3d)*sin(0.0175*conj(q2) - 1.5708) - 0.0175*cos(0.0175*conj(q1) - 1.5708)*cos(0.0175*conj(q2) - 1.5708)*conj(q2d)*(conj(q3) + conj(L2)) + 0.0175*cos(0.0175*conj(q1) - 1.5708)*cos(0.0175*conj(q2) - 1.5708)*conj(q2d)*(conj(q3) + conj(L2)) + 0.0175*conj(q1d)*sin(0.0175*conj(q1) - 1.5708)*sin(0.0175*conj(q2) - 1.5708)*(conj(q3) + conj(L2)) - 0.0175*conj(q1d)*sin(0.0175*conj(q1) - 1.5708)*sin(0.0175*conj(q2) - 1.5708)*(conj(q3) + conj(L2)) - 0.0175*cos(0.0175*conj(q1) - 1.5708)*cos(0.0175*conj(q2) - 1.5708)*conj(q2d)*conj(L3) + 0.0175*cos(0.0175*conj(q1) - 1.5708)*cos(0.0175*conj(q2) - 1.5708)*conj(q2d)*conj(L3) + 0.0175*conj(q1d)*sin(0.0175*conj(q1) - 1.5708)*sin(0.0175*conj(q2) - 1.5708)*conj(L3) - 0.0175*conj(q1d)*sin(0.0175*conj(q1) - 1.5708)*sin(0.0175*conj(q2) - 1.5708)*conj(L3)), (sin(0.0175*conj(q5) + 1.5708)*(cos(0.0175*conj(q1) - 1.5708)*sin(0.0175*conj(q4) + 1.5708) + cos(0.0175*conj(q2) - 1.5708)*cos(0.0175*conj(q4) + 1.5708)*sin(0.0175*conj(q1) - 1.5708)) - cos(0.0175*conj(q5) + 1.5708)*sin(0.0175*conj(q1) - 1.5708)*sin(0.0175*conj(q2) - 1.5708))*(conj(L4)*(sin(0.0175*conj(q5) + 1.5708)*(0.0175*cos(0.0175*conj(q1) - 1.5708)*conj(q1d)*sin(0.0175*conj(q4) + 1.5708) + 0.0175*cos(0.0175*conj(q4) + 1.5708)*conj(q4d)*sin(0.0175*conj(q1) - 1.5708) + 0.0175*cos(0.0175*conj(q2) - 1.5708)*cos(0.0175*conj(q4) + 1.5708)*conj(q1d)*sin(0.0175*conj(q1) - 1.5708) + 0.0175*cos(0.0175*conj(q1) - 1.5708)*cos(0.0175*conj(q4) + 1.5708)*conj(q2d)*sin(0.0175*conj(q2) - 1.5708) + 0.0175*cos(0.0175*conj(q1) - 1.5708)*cos(0.0175*conj(q2) - 1.5708)*conj(q4d)*sin(0.0175*conj(q4) + 1.5708)) + 0.0175*cos(0.0175*conj(q5) + 1.5708)*conj(q5d)*(sin(0.0175*conj(q1) - 1.5708)*sin(0.0175*conj(q4) + 1.5708) - cos(0.0175*conj(q1) - 1.5708)*cos(0.0175*conj(q2) - 1.5708)*cos(0.0175*conj(q4) + 1.5708)) + 0.0175*cos(0.0175*conj(q1) - 1.5708)*cos(0.0175*conj(q2) - 1.5708)*cos(0.0175*conj(q5) + 1.5708)*conj(q2d) - 0.0175*cos(0.0175*conj(q5) + 1.5708)*conj(q1d)*sin(0.0175*conj(q1) - 1.5708)*sin(0.0175*conj(q2) - 1.5708) - 0.0175*cos(0.0175*conj(q1) - 1.5708)*conj(q5d)*sin(0.0175*conj(q2) - 1.5708)*sin(0.0175*conj(q5) + 1.5708)) - cos(0.0175*conj(q1) - 1.5708)*conj(q3d)*sin(0.0175*conj(q2) - 1.5708) + cos(0.0175*conj(q1) - 1.5708)*conj(q3d)*sin(0.0175*conj(q2) - 1.5708) - 0.0175*cos(0.0175*conj(q1) - 1.5708)*cos(0.0175*conj(q2) - 1.5708)*conj(q2d)*(conj(q3) + conj(L2)) + 0.0175*cos(0.0175*conj(q1) - 1.5708)*cos(0.0175*conj(q2) - 1.5708)*conj(q2d)*(conj(q3) + conj(L2)) + 0.0175*conj(q1d)*sin(0.0175*conj(q1) - 1.5708)*sin(0.0175*conj(q2) - 1.5708)*(conj(q3) + conj(L2)) - 0.0175*conj(q1d)*sin(0.0175*conj(q1) - 1.5708)*sin(0.0175*conj(q2) - 1.5708)*(conj(q3) + conj(L2)) - 0.0175*cos(0.0175*conj(q1) - 1.5708)*cos(0.0175*conj(q2) - 1.5708)*conj(q2d)*conj(L3) + 0.0175*cos(0.0175*conj(q1) - 1.5708)*cos(0.0175*conj(q2) - 1.5708)*conj(q2d)*conj(L3) + 0.0175*conj(q1d)*sin(0.0175*conj(q1) - 1.5708)*sin(0.0175*conj(q2) - 1.5708)*conj(L3) - 0.0175*conj(q1d)*sin(0.0175*conj(q1) - 1.5708)*sin(0.0175*conj(q2) - 1.5708)*conj(L3)) - (conj(L4)*(sin(0.0175*conj(q5) + 1.5708)*(sin(0.0175*conj(q1) - 1.5708)*sin(0.0175*conj(q4) + 1.5708) - cos(0.0175*conj(q1) - 1.5708)*cos(0.0175*conj(q2) - 1.5708)*cos(0.0175*conj(q4) + 1.5708)) + cos(0.0175*conj(q1) - 1.5708)*cos(0.0175*conj(q5) + 1.5708)*sin(0.0175*conj(q2) - 1.5708)) - cos(0.0175*conj(q1) - 1.5708)*sin(0.0175*conj(q2) - 1.5708)*conj(L3) + cos(0.0175*conj(q1) - 1.5708)*sin(0.0175*conj(q2) - 1.5708)*conj(L3) - cos(0.0175*conj(q1) - 1.5708)*sin(0.0175*conj(q2) - 1.5708)*(conj(q3) + conj(L2)) + cos(0.0175*conj(q1) - 1.5708)*sin(0.0175*conj(q2) - 1.5708)*(conj(q3) + conj(L2)))*(sin(0.0175*conj(q5) + 1.5708)*(0.0175*conj(q1d)*sin(0.0175*conj(q1) - 1.5708)*sin(0.0175*conj(q4) + 1.5708) - 0.0175*cos(0.0175*conj(q1) - 1.5708)*cos(0.0175*conj(q4) + 1.5708)*conj(q4d) - 0.0175*cos(0.0175*conj(q1) - 1.5708)*cos(0.0175*conj(q2) - 1.5708)*cos(0.0175*conj(q4) + 1.5708)*conj(q1d) + 0.0175*cos(0.0175*conj(q4) + 1.5708)*conj(q2d)*sin(0.0175*conj(q1) - 1.5708)*sin(0.0175*conj(q2) - 1.5708) + 0.0175*cos(0.0175*conj(q2) - 1.5708)*conj(q4d)*sin(0.0175*conj(q1) - 1.5708)*sin(0.0175*conj(q4) + 1.5708)) - 0.0175*cos(0.0175*conj(q5) + 1.5708)*conj(q5d)*(cos(0.0175*conj(q1) - 1.5708)*sin(0.0175*conj(q4) + 1.5708) + cos(0.0175*conj(q2) - 1.5708)*cos(0.0175*conj(q4) + 1.5708)*sin(0.0175*conj(q1) - 1.5708)) + 0.0175*cos(0.0175*conj(q1) - 1.5708)*cos(0.0175*conj(q5) + 1.5708)*conj(q1d)*sin(0.0175*conj(q2) - 1.5708) + 0.0175*cos(0.0175*conj(q2) - 1.5708)*cos(0.0175*conj(q5) + 1.5708)*conj(q2d)*sin(0.0175*conj(q1) - 1.5708) - 0.0175*conj(q5d)*sin(0.0175*conj(q1) - 1.5708)*sin(0.0175*conj(q2) - 1.5708)*sin(0.0175*conj(q5) + 1.5708)) - (conj(L4)*(sin(0.0175*conj(q5) + 1.5708)*(cos(0.0175*conj(q1) - 1.5708)*sin(0.0175*conj(q4) + 1.5708) + cos(0.0175*conj(q2) - 1.5708)*cos(0.0175*conj(q4) + 1.5708)*sin(0.0175*conj(q1) - 1.5708)) - cos(0.0175*conj(q5) + 1.5708)*sin(0.0175*conj(q1) - 1.5708)*sin(0.0175*conj(q2) - 1.5708)) + sin(0.0175*conj(q1) - 1.5708)*sin(0.0175*conj(q2) - 1.5708)*(conj(q3) + conj(L2)) - sin(0.0175*conj(q1) - 1.5708)*sin(0.0175*conj(q2) - 1.5708)*(conj(q3) + conj(L2)) + sin(0.0175*conj(q1) - 1.5708)*sin(0.0175*conj(q2) - 1.5708)*conj(L3) - sin(0.0175*conj(q1) - 1.5708)*sin(0.0175*conj(q2) - 1.5708)*conj(L3))*(sin(0.0175*conj(q5) + 1.5708)*(0.0175*cos(0.0175*conj(q1) - 1.5708)*conj(q1d)*sin(0.0175*conj(q4) + 1.5708) + 0.0175*cos(0.0175*conj(q4) + 1.5708)*conj(q4d)*sin(0.0175*conj(q1) - 1.5708) + 0.0175*cos(0.0175*conj(q2) - 1.5708)*cos(0.0175*conj(q4) + 1.5708)*conj(q1d)*sin(0.0175*conj(q1) - 1.5708) + 0.0175*cos(0.0175*conj(q1) - 1.5708)*cos(0.0175*conj(q4) + 1.5708)*conj(q2d)*sin(0.0175*conj(q2) - 1.5708) + 0.0175*cos(0.0175*conj(q1) - 1.5708)*cos(0.0175*conj(q2) - 1.5708)*conj(q4d)*sin(0.0175*conj(q4) + 1.5708)) + 0.0175*cos(0.0175*conj(q5) + 1.5708)*conj(q5d)*(sin(0.0175*conj(q1) - 1.5708)*sin(0.0175*conj(q4) + 1.5708) - cos(0.0175*conj(q1) - 1.5708)*cos(0.0175*conj(q2) - 1.5708)*cos(0.0175*conj(q4) + 1.5708)) + 0.0175*cos(0.0175*conj(q1) - 1.5708)*cos(0.0175*conj(q2) - 1.5708)*cos(0.0175*conj(q5) + 1.5708)*conj(q2d) - 0.0175*cos(0.0175*conj(q5) + 1.5708)*conj(q1d)*sin(0.0175*conj(q1) - 1.5708)*sin(0.0175*conj(q2) - 1.5708) - 0.0175*cos(0.0175*conj(q1) - 1.5708)*conj(q5d)*sin(0.0175*conj(q2) - 1.5708)*sin(0.0175*conj(q5) + 1.5708)) + (sin(0.0175*conj(q5) + 1.5708)*(sin(0.0175*conj(q1) - 1.5708)*sin(0.0175*conj(q4) + 1.5708) - cos(0.0175*conj(q1) - 1.5708)*cos(0.0175*conj(q2) - 1.5708)*cos(0.0175*conj(q4) + 1.5708)) + cos(0.0175*conj(q1) - 1.5708)*cos(0.0175*conj(q5) + 1.5708)*sin(0.0175*conj(q2) - 1.5708))*(conj(L4)*(sin(0.0175*conj(q5) + 1.5708)*(0.0175*conj(q1d)*sin(0.0175*conj(q1) - 1.5708)*sin(0.0175*conj(q4) + 1.5708) - 0.0175*cos(0.0175*conj(q1) - 1.5708)*cos(0.0175*conj(q4) + 1.5708)*conj(q4d) - 0.0175*cos(0.0175*conj(q1) - 1.5708)*cos(0.0175*conj(q2) - 1.5708)*cos(0.0175*conj(q4) + 1.5708)*conj(q1d) + 0.0175*cos(0.0175*conj(q4) + 1.5708)*conj(q2d)*sin(0.0175*conj(q1) - 1.5708)*sin(0.0175*conj(q2) - 1.5708) + 0.0175*cos(0.0175*conj(q2) - 1.5708)*conj(q4d)*sin(0.0175*conj(q1) - 1.5708)*sin(0.0175*conj(q4) + 1.5708)) - 0.0175*cos(0.0175*conj(q5) + 1.5708)*conj(q5d)*(cos(0.0175*conj(q1) - 1.5708)*sin(0.0175*conj(q4) + 1.5708) + cos(0.0175*conj(q2) - 1.5708)*cos(0.0175*conj(q4) + 1.5708)*sin(0.0175*conj(q1) - 1.5708)) + 0.0175*cos(0.0175*conj(q1) - 1.5708)*cos(0.0175*conj(q5) + 1.5708)*conj(q1d)*sin(0.0175*conj(q2) - 1.5708) + 0.0175*cos(0.0175*conj(q2) - 1.5708)*cos(0.0175*conj(q5) + 1.5708)*conj(q2d)*sin(0.0175*conj(q1) - 1.5708) - 0.0175*conj(q5d)*sin(0.0175*conj(q1) - 1.5708)*sin(0.0175*conj(q2) - 1.5708)*sin(0.0175*conj(q5) + 1.5708)) - conj(q3d)*sin(0.0175*conj(q1) - 1.5708)*sin(0.0175*conj(q2) - 1.5708) + conj(q3d)*sin(0.0175*conj(q1) - 1.5708)*sin(0.0175*conj(q2) - 1.5708) - 0.0175*cos(0.0175*conj(q1) - 1.5708)*conj(q1d)*sin(0.0175*conj(q2) - 1.5708)*(conj(q3) + conj(L2)) - 0.0175*cos(0.0175*conj(q2) - 1.5708)*conj(q2d)*sin(0.0175*conj(q1) - 1.5708)*(conj(q3) + conj(L2)) + 0.0175*cos(0.0175*conj(q1) - 1.5708)*conj(q1d)*sin(0.0175*conj(q2) - 1.5708)*(conj(q3) + conj(L2)) + 0.0175*cos(0.0175*conj(q2) - 1.5708)*conj(q2d)*sin(0.0175*conj(q1) - 1.5708)*(conj(q3) + conj(L2)) - 0.0175*cos(0.0175*conj(q1) - 1.5708)*conj(q1d)*sin(0.0175*conj(q2) - 1.5708)*conj(L3) - 0.0175*cos(0.0175*conj(q2) - 1.5708)*conj(q2d)*sin(0.0175*conj(q1) - 1.5708)*conj(L3) + 0.0175*cos(0.0175*conj(q1) - 1.5708)*conj(q1d)*sin(0.0175*conj(q2) - 1.5708)*conj(L3) + 0.0175*cos(0.0175*conj(q2) - 1.5708)*conj(q2d)*sin(0.0175*conj(q1) - 1.5708)*conj(L3));
                                                                                                                                                                                                                                                                                                                                                                                                                                                                                                                                                                                                                                                                                                                                                                                                                                                                                                                                                                                                                                                                                                                                                                                                                                                                                                                                                                                                                                                                                                                                                                                                                                                                                                                                                                                                                                                      0,                                                                                                                                                                                                                                                                                                                                                                                                                                                                                                                                                                                                                                                                                                                                                                                                                                                                                                                                                                                                                                                                                                                                                                                                                                                                                                                                                                                                                                                                                                                                                                                                                                                                                                                                                                                                                                                                                                                                                                                                                                                                                                                                                                                                                                                                                                                                                                                                                                                                                                                                                                                                                                                                                                                                                                                                                                                                                                                                                                                                                                                                                                                                                                                                                                                                                                                                                                                                                                                                                                                                                                                                                                                                                                                                                                                                                                                                                                                                                                                                                                                                                                                                                                                                                                                                                                                                                                                                                                                                                                                                                                                                                                                                                                                                                                                                                                                                               -0.0175*cos(0.0175*q1 - 1.5708)*q1d,                                                                                                                                                         0,                                                                                                                                                                                                                                                                                                                                                                                                                                                                                                                                                                                                                                                                                                                                                                                                                                                                                                                                                                                                                                                                                                                                                                                                                                                                                                                                                                                                                                                                                                                                                                                                                                                                                                                                                                                                                                                                                                                                                                                                                                                                                                                                                                                                                                                                                                                                                                                                                                                                                                                                                                                                                                                                                                                                                                                                                                                                                                                                                                                                                                                                                                                                                                                                                                                                                                                                                                                                                                                                                                                                                                                                                                                                                                                                                                                                                                                                                                                                                                                                                                                                                                                                                                                                                                                                                                                                                                                                                                                                                                                                                                                                                                                                                                                                                                                                                                                                                                                                                                                                                                                                                                                                                                                                                                                                                                                                                                                                                                                                                                                                                                                                                                                                                                                                                                                                                                                                                                                                                                                                                                                                                                                                                                                                                                                                                                                                                                                                                                                                                                                                                                                                                                                                                                                                                                                                                                                                                                                                                                                                                                                                                                                                                                                                 0.0175*cos(0.0175*q1 - 1.5708)*cos(0.0175*q2 - 1.5708)*q2d - 0.0175*sin(0.0175*q1 - 1.5708)*sin(0.0175*q2 - 1.5708)*q1d,                                                                                                                                                                                                                                                                                                                                                                                                                                                                                                                                                                                                                                                                                                                                                                                                                                                                                                                                                                                                                                                                                                                                                                                                                                                                                                                                                                                                                                                                                                                                                                                                                                                                                                                                                                                                                                                                                                                                                                                                                                                                                                                                                                                                                                                                                                                                                                                                                                                                                                                                                                                                                                                                                                                                                                                                                                                                                                                                                                                                                                                                                                                                                                                                                                                                                                                                                                                                                                                                                                                                                                                                                                                                                                                                                                                                                                                                                                                                                                                                                                                                                                                                                                                                                                                                                                                                                                                                                                                                                                                                                                                                                                                                                                                                                                                                                                                                                                                                                                                                                                                                                                                                                                                                                                                                                                                                                                                                                                                                                                                                                                                                                                                                                                                                                                                                                                                                                                                                                                                                                                                                                                                                                                                                                                                                                                                                                                                                                                                                                                                                                                                                                                                                                                                                                                                                                                                                                                                                                                                                                                                                                                                                                                                                                                                                                      0.0175*cos(0.0175*q1 - 1.5708)*cos(0.0175*q4 + 1.5708)*q1d - 0.0175*sin(0.0175*q1 - 1.5708)*sin(0.0175*q4 + 1.5708)*q4d + 0.0175*cos(0.0175*q1 - 1.5708)*cos(0.0175*q2 - 1.5708)*cos(0.0175*q4 + 1.5708)*q4d - 0.0175*cos(0.0175*q2 - 1.5708)*sin(0.0175*q1 - 1.5708)*sin(0.0175*q4 + 1.5708)*q1d - 0.0175*cos(0.0175*q1 - 1.5708)*sin(0.0175*q2 - 1.5708)*sin(0.0175*q4 + 1.5708)*q2d,                                                                                                                                                                                                                                                                                                                                                                                                                                                                                                                                                                                                                                                                                                                                                                                                                                                                                                                                                                                                                                                                                                                                                                                                                                                                                                                                                                                                                                                                                                                                                                                                                                                                                                                                                                                                                                                                                                                                                                                                                                                                                                                                                                                                                                                                                                                                                                                                                                                                                                                                                                                                                                                                                                                                                                                                                                                                                                                                                                                                                                                                                                                                                                                                                                                                                                                                                                                                                                                                                                                                                                                                                                                                                                                                                                                                                                                                                                                                                                                                                                                                                                                                                                                                                                                                                                                                                                                                                                                                                                                                                                                                                                                                                                                                                                                                                                                                                                                                                                                                                                                                                                                                                                                                                                                                                                                                                                                                                                                                                                                                                                                                                                                                                                                                                                                                                                                                                                                                                                                                                                                                                                                                                                                                                                                                                                                                                                                                                                                                                                                                                                                                                                                                                                                                                                                                                                                                                                                                                                                                                                                                                                                                                                                                                                                                                                                                                                                                                                                                                                                                                                                                                                                                                                                                                                                                                                                                                                                                                                                                                                                                                                                                                                                                                                                                                                                                                                            0.0175*cos(0.0175*q5 + 1.5708)*sin(0.0175*q1 - 1.5708)*sin(0.0175*q2 - 1.5708)*q1d - 0.0175*cos(0.0175*q5 + 1.5708)*q5d*(sin(0.0175*q1 - 1.5708)*sin(0.0175*q4 + 1.5708) - cos(0.0175*q1 - 1.5708)*cos(0.0175*q2 - 1.5708)*cos(0.0175*q4 + 1.5708)) - 0.0175*cos(0.0175*q1 - 1.5708)*cos(0.0175*q2 - 1.5708)*cos(0.0175*q5 + 1.5708)*q2d - sin(0.0175*q5 + 1.5708)*(0.0175*cos(0.0175*q1 - 1.5708)*sin(0.0175*q4 + 1.5708)*q1d + 0.0175*cos(0.0175*q4 + 1.5708)*sin(0.0175*q1 - 1.5708)*q4d + 0.0175*cos(0.0175*q2 - 1.5708)*cos(0.0175*q4 + 1.5708)*sin(0.0175*q1 - 1.5708)*q1d + 0.0175*cos(0.0175*q1 - 1.5708)*cos(0.0175*q4 + 1.5708)*sin(0.0175*q2 - 1.5708)*q2d + 0.0175*cos(0.0175*q1 - 1.5708)*cos(0.0175*q2 - 1.5708)*sin(0.0175*q4 + 1.5708)*q4d) + 0.0175*cos(0.0175*q1 - 1.5708)*sin(0.0175*q2 - 1.5708)*sin(0.0175*q5 + 1.5708)*q5d;
